simulink model "Hospital"  (R2022b)
settings: Solver=VariableStepAuto  StartTime=0.0  StopTime=10.0  RelTol=1e-3
(part 1 of 2)
settings Model: Creator=Stefano  LastModifiedBy=stefanopanzieri
settings SolverCC: AlgebraicLoopSolver=TrustRegion
settings DebuggingCC: UnconnectedInputMsg=warning  UnconnectedOutputMsg=warning  UnconnectedLineMsg=warning  SFMachineParentedDataDiag=warning
settings ModelReferenceCC: EnableRefExpFcnMdlSchedulingChecks=on
settings SFSimCC: CustomCodeUndefinedFunction=UseInterfaceOnly
settings RTWCC: DLArmComputeVersion=19.05

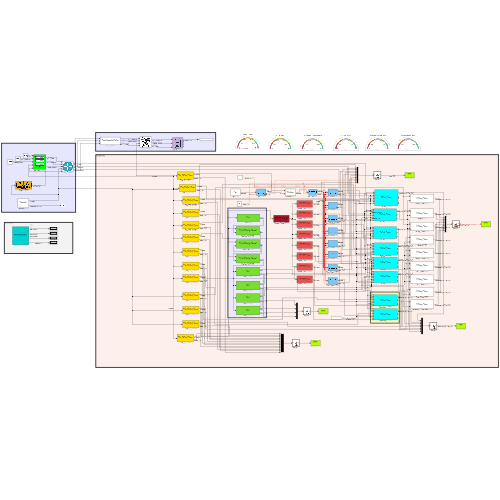
[thumbnail: Simulink's stored preview of the top-level diagram]
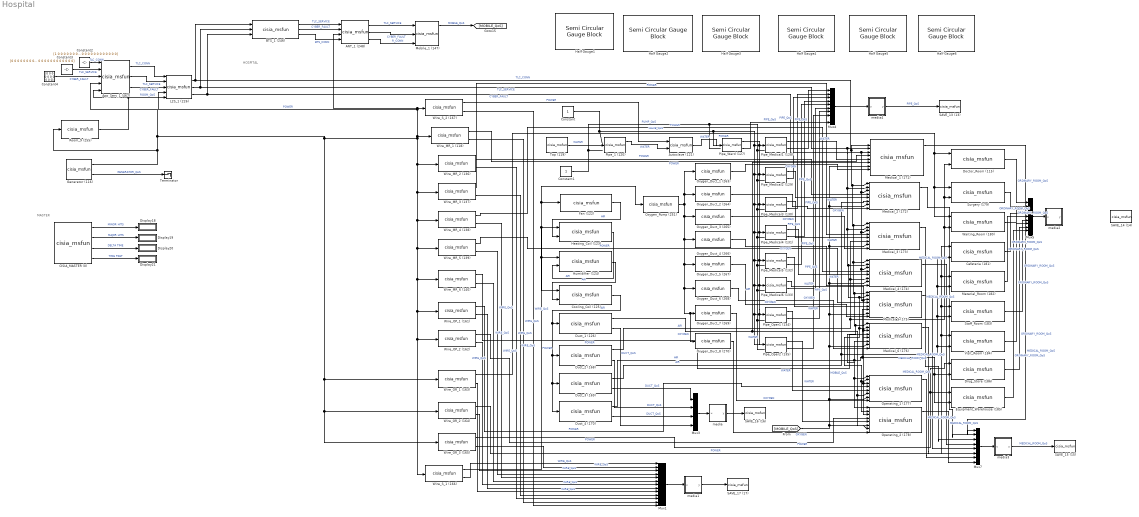
== system Hospital ==
  note: HOSPITAL
  note: MASTER
  ANT_1 (248) : M-S-Function  FunctionName=cisia_msfun  Parameters=Parameter1, Parameter2, Parameter3, resources, Parameter10, codeupdate, step_received, step_computed, dynamic_computed, step_sended, id_entity, id_project, id_type, name_type, color  mask(S-function:msfcn_unit_delay){Parameter1='ANT_1', Parameter2=1, Parameter3='ORO', resources=, Parameter10=off, codeupdate=off, step_received=|, step_computed=, dynamic_computed=, step_sended=|, id_entity=427, id_project=6, id_type=55, name_type=BTS_ANTENNA, color=#FFFFFF}
      mask step_received=|
      | Connection=max(Connection_init,BTS_CONN);
      | TLC_services=max(TLC_services_init,TLC_SERVICE);
      | TLC_services=mod(TLC_services,10);
      | TLC_revoke=floor(TLC_SERVICE/10);
      |
      | Cyber_Fault=max(CYBER_FAULT, transpose([Dos_attack   MITM_attack Virus_Attack Port_Scan_Attack  BGP_hijacking BotNet_Attack Data_Corruption SW_Change Config_Change Port_Saturation]));
      |
      | Conn_Fault=max([Dos_attack  Mechanical_Fault  1-POWER] );
      |
      | Service_Fault=max(abs(Consumed_Services.*TLC_services-Consumed_Services));
      | Redundancy_Fault=max(abs(Consumed_Services.*BTS_CONN-Consumed_Services));
      |
      | Operative_Level=(1-Conn_Fault)*(1-0.5*max(Cyber_Fault))*(1-Service_Fault);
      |
      | %Operative_Level=(1-Conn_Fault)*((2*(1-Service_Fault)+(1-Redundancy_Fault))/3);
      | %Operative_Level=(1-Conn_Fault)*max(max(BTS_CONN),0.5)*((2*(1-Service_Fault)+(1-Redundancy_Fault))/3);
      |
      | % Il servizio utilizzato
      | %My_Service=max([(1-Service_Fault) (1-Redundancy_Fault)/2]);
      mask step_sended=|
      | R_CONN=Connection*(1-Conn_Fault);
      | TLC_SERVICE=TLC_services*(1-Conn_Fault)*(1-Service_Fault)+10*TLC_revoke;
      | CYBER_FAULT=Cyber_Fault*(1-Conn_Fault);
      mask prompts: Parameter1 "entity name"; Parameter2 "sampling time"; Parameter3 "project"; resources "input resources and state variables"; Parameter10 "Bring state variables to output"; codeupdate "update code from mask"
      mask help: This is a level-2 MATLAB file S-function which demonstrates CISIA entity
      mask DialogControl Container1 Prompt: All parameters
      mask Display: image('Icons/BTS_ANTENNA.png')
  App_Serv_1 (467) : M-S-Function  FunctionName=cisia_msfun  Parameters=Parameter1, Parameter2, Parameter3, resources, Parameter10, codeupdate, step_received, step_computed, dynamic_computed, step_sended, id_entity, id_project, id_type, name_type, color  mask(S-function:msfcn_unit_delay){Parameter1='App_Serv_1', Parameter2=1, Parameter3='ORO', resources=, Parameter10=off, codeupdate=off, step_received=|, step_computed=, dynamic_computed=, step_sended=|, id_entity=467, id_project=6, id_type=40, name_type=App_Server, color=#00AAFF}
      mask step_received=|
      | Connection=max(Connection_init,TLC_CONN);
      | TLC_services=max(TLC_services_init,TLC_SERVICE);
      | TLC_services=mod(TLC_services,10);
      | TLC_revoke=floor(TLC_SERVICE/10);
      |
      | Mechanical_Fault=max([Mechanical_Fault Mechanical_Fault_init]);
      |
      | %if strcmp(name_entity,"BlockChainServer") && (cisia.major_time>=2)
      |  % Dos_attack=1;
      |  %TLC_revoke(9)=1;
      |  %TLC_services(9)=0;
      | %end
      |
      |
      | Cyber_Fault=max(CYBER_FAULT, transpose([Dos_attack   MITM_attack Virus_Attack Port_Scan_Attack  BGP_hijacking BotNet_Attack Data_Corruption SW_Change Config_Change Port_Saturation]));
      |
      | Service_Fault=max(abs(Consumed_Services.*TLC_services-Consumed_Services));
      | Redundancy_Fault=max(abs(Consumed_Services.*TLC_CONN-Consumed_Services));
      |
      | Conn_Fault=max([Dos_attack  Mechanical_Fault  1-POWER 1-ROOM_QoS] );
      |
      |
      | Operative_Level=(1-Conn_Fault)*(1-0.5*max(Cyber_Fault))*(1-Service_Fault)*max(max(TLC_CONN),0.5);
      mask step_sended=|
      | TLC_CONN=Connection*(1-Conn_Fault);
      | TLC_SERVICE=TLC_services*(1-Conn_Fault)*(1-Service_Fault)*(1-syslog_adm_login)+10*TLC_revoke;
      | CYBER_FAULT=Cyber_Fault*(1-Conn_Fault);
      mask prompts: Parameter1 "entity name"; Parameter2 "sampling time"; Parameter3 "project"; resources "input resources and state variables"; Parameter10 "Bring state variables to output"; codeupdate "update code from mask"
      mask help: This is a level-2 MATLAB file S-function which demonstrates CISIA entity
      mask DialogControl Container1 Prompt: All parameters
      mask Display: image('Icons/App_Server.png')
  Autoclave (121) : M-S-Function  FunctionName=cisia_msfun  Parameters=Parameter1, Parameter2, Parameter3, resources, Parameter10, codeupdate, step_received, step_computed, dynamic_computed, step_sended, id_entity, id_project, id_type, name_type, color  mask(S-function:msfcn_unit_delay){Parameter1='Autoclave', Parameter2=1, Parameter3='ORO', resources=, Parameter10=off, codeupdate=off, step_received=|, step_computed=, dynamic_computed=, step_sended=WATER=Operative_Level;, id_entity=425, id_project=6, id_type=33, name_type=Autoclave, color=#FFFFFF}
      mask step_received=|
      | Water_Fault=1-WATER;
      | Power_Fault=1-POWER;
      |
      | Operative_Level=min([ 1-Mechanical_Fault 1-Power_Fault 1-Water_Fault]);
      mask prompts: Parameter1 "entity name"; Parameter2 "sampling time"; Parameter3 "project"; resources "input resources and state variables"; Parameter10 "Bring state variables to output"; codeupdate "update code from mask"
      mask help: This is a level-2 MATLAB file S-function which demonstrates CISIA entity
      mask DialogControl Container1 Prompt: All parameters
      mask Display: disp('Autoclave')
  BTS_1 (246) : M-S-Function  FunctionName=cisia_msfun  Parameters=Parameter1, Parameter2, Parameter3, resources, Parameter10, codeupdate, step_received, step_computed, dynamic_computed, step_sended, id_entity, id_project, id_type, name_type, color  mask(S-function:msfcn_unit_delay){Parameter1='BTS_1', Parameter2=1, Parameter3='ORO', resources=, Parameter10=off, codeupdate=off, step_received=|, step_computed=, dynamic_computed=, step_sended=|, id_entity=428, id_project=6, id_type=54, name_type=BaseTransceiverStation, color=#FFFFFF}
      mask step_received=|
      | Connection=max(Connection_init,TLC_CONN);
      | TLC_services=max(TLC_services_init,TLC_SERVICE);
      | TLC_services=mod(TLC_services,10);
      | TLC_revoke=floor(TLC_SERVICE/10);
      |
      | Cyber_Fault=max(CYBER_FAULT, transpose([Dos_attack   MITM_attack Virus_Attack Port_Scan_Attack  BGP_hijacking BotNet_Attack Data_Corruption SW_Change Config_Change Port_Saturation]));
      |
      | Conn_Fault=max([Dos_attack  Mechanical_Fault ] );
      |
      | Operative_Level=(1-Conn_Fault)*max(max(TLC_services),0.5)*(1-0.5*max(Cyber_Fault));
      mask step_sended=|
      | BTS_CONN=Connection*(1-Conn_Fault);
      | TLC_SERVICE=TLC_services*(1-Conn_Fault)+10*TLC_revoke;
      | CYBER_FAULT=Cyber_Fault*(1-Conn_Fault);
      mask prompts: Parameter1 "entity name"; Parameter2 "sampling time"; Parameter3 "project"; resources "input resources and state variables"; Parameter10 "Bring state variables to output"; codeupdate "update code from mask"
      mask help: This is a level-2 MATLAB file S-function which demonstrates CISIA entity
      mask DialogControl Container1 Prompt: All parameters
      mask Display: disp('BaseTransceiverStation')
  CISIA_MASTER (0) : M-S-Function  FunctionName=cisia_msfun  Parameters=Parameter1, Parameter2, Parameter3, resources, Parameter4, Parameter5, Parameter6, Parameter7, Parameter8, Parameter9,Parameter11  mask(S-function:msfcn_unit_delay){Parameter1='CISIA_MASTER', Parameter2=1, Parameter3='SistemiIoT', resources=off, Parameter4=on, Parameter5=off, Parameter6=off, Parameter7=off, Parameter8=0.001, Parameter9=off, Parameter11=on}
      mask prompts: Parameter1 "entity name"; Parameter2 "sampling time"; Parameter3 "project"; resources "Save status at each major hit"; Parameter4 "Show Operative Levels with colors"; Parameter5 "Load Entities from file"; Parameter6 "Load Start from Mask"; Parameter7 "Real Time"; Parameter8 "Real Time Hit (sec)"; Parameter9 "Skip saving"; Parameter11 "Show unconnected"
      mask help: This is a level-2 MATLAB file S-function which demonstrates CISIA entity
      mask Display: disp('MASTER BLOCK')
  Cafeteria (181) : M-S-Function  FunctionName=cisia_msfun  Parameters=Parameter1, Parameter2, Parameter3, resources, Parameter10, codeupdate, step_received, step_computed, dynamic_computed, step_sended, id_entity, id_project, id_type, name_type, color  mask(S-function:msfcn_unit_delay){Parameter1='Cafeteria', Parameter2=1, Parameter3='ORO', resources=, Parameter10=off, codeupdate=off, step_received=|, step_computed=, dynamic_computed=, step_sended=ORDINARY_ROOM_QoS= Operative_Level;, id_entity=385, id_project=6, id_type=26, name_type=Ordinary_Room, color=#FFFFFF}
      mask step_received=|
      | Power_Fault=1-POWER;
      | Air_Fault=1-AIR;
      |
      |
      | Operative_Level=(1-Fire_Fault)*(1-0.5*Power_Fault)*(1-0-5*Air_Fault);
      mask prompts: Parameter1 "entity name"; Parameter2 "sampling time"; Parameter3 "project"; resources "input resources and state variables"; Parameter10 "Bring state variables to output"; codeupdate "update code from mask"
      mask help: This is a level-2 MATLAB file S-function which demonstrates CISIA entity
      mask DialogControl Container1 Prompt: All parameters
      mask Display: disp('Ordinary_Room')
  Constant : Constant
  Constant1 : Constant
  Constant2 : Constant  Value=[1 0 0 0 0 0 0 0 0 0 0 0 0 0 0 0 0 0 0 0]
  Constant3 : Constant  Value=[0 0 0 0 0 0 0 0 0 0 0 0 0 0 0 0 0 0 0 0]
  Constant4 : Constant  Value=[0 0 0 0 0 0 0 0 0 0]
  Cooling_Coil (125) : M-S-Function  FunctionName=cisia_msfun  Parameters=Parameter1, Parameter2, Parameter3, resources, Parameter10, codeupdate, step_received, step_computed, dynamic_computed, step_sended, id_entity, id_project, id_type, name_type, color  mask(S-function:msfcn_unit_delay){Parameter1='Cooling_Coil', Parameter2=1, Parameter3='ORO', resources=, Parameter10=off, codeupdate=off, step_received=|, step_computed=, dynamic_computed=, step_sended=AIR=Operative_Level;, id_entity=395, id_project=6, id_type=35, name_type=Air_Conditioning_Element, color=#79DE31}
      mask step_received=|
      | Power_Fault=1-POWER;
      | Air_Fault=1-AIR;
      |
      | Operative_Level=min([1-Mechanical_Fault 1-Power_Fault 1-Air_Fault]);
      mask prompts: Parameter1 "entity name"; Parameter2 "sampling time"; Parameter3 "project"; resources "input resources and state variables"; Parameter10 "Bring state variables to output"; codeupdate "update code from mask"
      mask help: This is a level-2 MATLAB file S-function which demonstrates CISIA entity
      mask DialogControl Container1 Prompt: All parameters
      mask Display: disp('Air_Conditioning_Element')
  Display{18..21} (4 alike) : Display
  Doctor_Room (115) : M-S-Function  FunctionName=cisia_msfun  Parameters=Parameter1, Parameter2, Parameter3, resources, Parameter10, codeupdate, step_received, step_computed, dynamic_computed, step_sended, id_entity, id_project, id_type, name_type, color  mask(S-function:msfcn_unit_delay){Parameter1='Doctor_Room', Parameter2=1, Parameter3='ORO', resources=, Parameter10=off, codeupdate=off, step_received=|, step_computed=, dynamic_computed=, step_sended=ORDINARY_ROOM_QoS= Operative_Level;, id_entity=414, id_project=6, id_type=26, name_type=Ordinary_Room, color=#FFFFFF}
      mask step_received=|
      | Power_Fault=1-POWER;
      | Air_Fault=1-AIR;
      |
      |
      | Operative_Level=(1-Fire_Fault)*(1-0.5*Power_Fault)*(1-0-5*Air_Fault);
      mask prompts: Parameter1 "entity name"; Parameter2 "sampling time"; Parameter3 "project"; resources "input resources and state variables"; Parameter10 "Bring state variables to output"; codeupdate "update code from mask"
      mask help: This is a level-2 MATLAB file S-function which demonstrates CISIA entity
      mask DialogControl Container1 Prompt: All parameters
      mask Display: disp('Ordinary_Room')
  Drug_Store (186) : M-S-Function  FunctionName=cisia_msfun  Parameters=Parameter1, Parameter2, Parameter3, resources, Parameter10, codeupdate, step_received, step_computed, dynamic_computed, step_sended, id_entity, id_project, id_type, name_type, color  mask(S-function:msfcn_unit_delay){Parameter1='Drug_Store', Parameter2=1, Parameter3='ORO', resources=, Parameter10=off, codeupdate=off, step_received=|, step_computed=, dynamic_computed=, step_sended=ORDINARY_ROOM_QoS= Operative_Level;, id_entity=389, id_project=6, id_type=26, name_type=Ordinary_Room, color=#FFFFFF}
      mask step_received=|
      | Power_Fault=1-POWER;
      | Air_Fault=1-AIR;
      |
      |
      | Operative_Level=(1-Fire_Fault)*(1-0.5*Power_Fault)*(1-0-5*Air_Fault);
      mask prompts: Parameter1 "entity name"; Parameter2 "sampling time"; Parameter3 "project"; resources "input resources and state variables"; Parameter10 "Bring state variables to output"; codeupdate "update code from mask"
      mask help: This is a level-2 MATLAB file S-function which demonstrates CISIA entity
      mask DialogControl Container1 Prompt: All parameters
      mask Display: disp('Ordinary_Room')
  Duct_1 (126) : M-S-Function  FunctionName=cisia_msfun  Parameters=Parameter1, Parameter2, Parameter3, resources, Parameter10, codeupdate, step_received, step_computed, dynamic_computed, step_sended, id_entity, id_project, id_type, name_type, color  mask(S-function:msfcn_unit_delay){Parameter1='Duct_1', Parameter2=1, Parameter3='ORO', resources=, Parameter10=off, codeupdate=off, step_received=|, step_computed=, dynamic_computed=, step_sended=|, id_entity=366, id_project=6, id_type=36, name_type=Duct, color=#79DE31}
      mask step_received=|
      | Air_Fault=1-AIR;
      |
      | Operative_Level=(1-Mechanical_Fault)*(1-0.5*Air_Fault);
      mask step_sended=|
      | AIR=Operative_Level;
      | DUCT_QoS=Operative_Level;
      mask prompts: Parameter1 "entity name"; Parameter2 "sampling time"; Parameter3 "project"; resources "input resources and state variables"; Parameter10 "Bring state variables to output"; codeupdate "update code from mask"
      mask help: This is a level-2 MATLAB file S-function which demonstrates CISIA entity
      mask DialogControl Container1 Prompt: All parameters
      mask Display: disp('Duct')
  Duct_2 (168) : M-S-Function  FunctionName=cisia_msfun  Parameters=Parameter1, Parameter2, Parameter3, resources, Parameter10, codeupdate, step_received, step_computed, dynamic_computed, step_sended, id_entity, id_project, id_type, name_type, color  mask(S-function:msfcn_unit_delay){Parameter1='Duct_2', Parameter2=1, Parameter3='ORO', resources=, Parameter10=off, codeupdate=off, step_received=|, step_computed=, dynamic_computed=, step_sended=|, id_entity=367, id_project=6, id_type=36, name_type=Duct, color=#79DE31}
      mask step_received=|
      | Air_Fault=1-AIR;
      |
      | Operative_Level=(1-Mechanical_Fault)*(1-0.5*Air_Fault);
      mask step_sended=|
      | AIR=Operative_Level;
      | DUCT_QoS=Operative_Level;
      mask prompts: Parameter1 "entity name"; Parameter2 "sampling time"; Parameter3 "project"; resources "input resources and state variables"; Parameter10 "Bring state variables to output"; codeupdate "update code from mask"
      mask help: This is a level-2 MATLAB file S-function which demonstrates CISIA entity
      mask DialogControl Container1 Prompt: All parameters
      mask Display: disp('Duct')
  Duct_3 (169) : M-S-Function  FunctionName=cisia_msfun  Parameters=Parameter1, Parameter2, Parameter3, resources, Parameter10, codeupdate, step_received, step_computed, dynamic_computed, step_sended, id_entity, id_project, id_type, name_type, color  mask(S-function:msfcn_unit_delay){Parameter1='Duct_3', Parameter2=1, Parameter3='ORO', resources=, Parameter10=off, codeupdate=off, step_received=|, step_computed=, dynamic_computed=, step_sended=|, id_entity=368, id_project=6, id_type=36, name_type=Duct, color=#79DE31}
      mask step_received=|
      | Air_Fault=1-AIR;
      |
      | Operative_Level=(1-Mechanical_Fault)*(1-0.5*Air_Fault);
      mask step_sended=|
      | AIR=Operative_Level;
      | DUCT_QoS=Operative_Level;
      mask prompts: Parameter1 "entity name"; Parameter2 "sampling time"; Parameter3 "project"; resources "input resources and state variables"; Parameter10 "Bring state variables to output"; codeupdate "update code from mask"
      mask help: This is a level-2 MATLAB file S-function which demonstrates CISIA entity
      mask DialogControl Container1 Prompt: All parameters
      mask Display: disp('Duct')
  Duct_4 (170) : M-S-Function  FunctionName=cisia_msfun  Parameters=Parameter1, Parameter2, Parameter3, resources, Parameter10, codeupdate, step_received, step_computed, dynamic_computed, step_sended, id_entity, id_project, id_type, name_type, color  mask(S-function:msfcn_unit_delay){Parameter1='Duct_4', Parameter2=1, Parameter3='ORO', resources=, Parameter10=off, codeupdate=off, step_received=|, step_computed=, dynamic_computed=, step_sended=|, id_entity=369, id_project=6, id_type=36, name_type=Duct, color=#79DE31}
      mask step_received=|
      | Air_Fault=1-AIR;
      |
      | Operative_Level=(1-Mechanical_Fault)*(1-0.5*Air_Fault);
      mask step_sended=|
      | AIR=Operative_Level;
      | DUCT_QoS=Operative_Level;
      mask prompts: Parameter1 "entity name"; Parameter2 "sampling time"; Parameter3 "project"; resources "input resources and state variables"; Parameter10 "Bring state variables to output"; codeupdate "update code from mask"
      mask help: This is a level-2 MATLAB file S-function which demonstrates CISIA entity
      mask DialogControl Container1 Prompt: All parameters
      mask Display: disp('Duct')
  Equipment_Warehouse (185) : M-S-Function  FunctionName=cisia_msfun  Parameters=Parameter1, Parameter2, Parameter3, resources, Parameter10, codeupdate, step_received, step_computed, dynamic_computed, step_sended, id_entity, id_project, id_type, name_type, color  mask(S-function:msfcn_unit_delay){Parameter1='Equipment_Warehouse', Parameter2=1, Parameter3='ORO', resources=, Parameter10=off, codeupdate=off, step_received=|, step_computed=, dynamic_computed=, step_sended=ORDINARY_ROOM_QoS= Operative_Level;, id_entity=390, id_project=6, id_type=26, name_type=Ordinary_Room, color=#FFFFFF}
      mask step_received=|
      | Power_Fault=1-POWER;
      | Air_Fault=1-AIR;
      |
      |
      | Operative_Level=(1-Fire_Fault)*(1-0.5*Power_Fault)*(1-0-5*Air_Fault);
      mask prompts: Parameter1 "entity name"; Parameter2 "sampling time"; Parameter3 "project"; resources "input resources and state variables"; Parameter10 "Bring state variables to output"; codeupdate "update code from mask"
      mask help: This is a level-2 MATLAB file S-function which demonstrates CISIA entity
      mask DialogControl Container1 Prompt: All parameters
      mask Display: disp('Ordinary_Room')
  Fan (122) : M-S-Function  FunctionName=cisia_msfun  Parameters=Parameter1, Parameter2, Parameter3, resources, Parameter10, codeupdate, step_received, step_computed, dynamic_computed, step_sended, id_entity, id_project, id_type, name_type, color  mask(S-function:msfcn_unit_delay){Parameter1='Fan', Parameter2=1, Parameter3='ORO', resources=, Parameter10=off, codeupdate=off, step_received=|, step_computed=, dynamic_computed=, step_sended=AIR=Operative_Level;, id_entity=391, id_project=6, id_type=34, name_type=Fan, color=#79DE31}
      mask step_received=|
      | Power_Fault=1-POWER;
      |
      | Operative_Level=(1-Mechanical_Fault)*(1-0.5*Power_Fault);
      mask prompts: Parameter1 "entity name"; Parameter2 "sampling time"; Parameter3 "project"; resources "input resources and state variables"; Parameter10 "Bring state variables to output"; codeupdate "update code from mask"
      mask help: This is a level-2 MATLAB file S-function which demonstrates CISIA entity
      mask DialogControl Container1 Prompt: All parameters
      mask Display: disp('Fan')
  Generator (116) : M-S-Function  FunctionName=cisia_msfun  Parameters=Parameter1, Parameter2, Parameter3, resources, Parameter10, codeupdate, step_received, step_computed, dynamic_computed, step_sended, id_entity, id_project, id_type, name_type, color  mask(S-function:msfcn_unit_delay){Parameter1='Generator', Parameter2=1, Parameter3='ORO', resources=, Parameter10=off, codeupdate=off, step_received=Operative_Level=1-Mechanical_Fault;, step_computed=, dynamic_computed=, step_sended=|, id_entity=392, id_project=6, id_type=27, name_type=Generator, color=#FFFFFF}
      mask step_sended=|
      | POWER=Operative_Level;
      | GENERATOR_QoS=Operative_Level;
      mask prompts: Parameter1 "entity name"; Parameter2 "sampling time"; Parameter3 "project"; resources "input resources and state variables"; Parameter10 "Bring state variables to output"; codeupdate "update code from mask"
      mask help: This is a level-2 MATLAB file S-function which demonstrates CISIA entity
      mask DialogControl Container1 Prompt: All parameters
      mask Display: disp('Generator')
  Half Gauge{1..6} (6 alike) : SemiCircularGaugeBlock  ScaleMax=1
  Heating_Coil (123) : M-S-Function  FunctionName=cisia_msfun  Parameters=Parameter1, Parameter2, Parameter3, resources, Parameter10, codeupdate, step_received, step_computed, dynamic_computed, step_sended, id_entity, id_project, id_type, name_type, color  mask(S-function:msfcn_unit_delay){Parameter1='Heating_Coil', Parameter2=1, Parameter3='ORO', resources=, Parameter10=off, codeupdate=off, step_received=|, step_computed=, dynamic_computed=, step_sended=AIR=Operative_Level;, id_entity=393, id_project=6, id_type=35, name_type=Air_Conditioning_Element, color=#79DE31}
      mask step_received=|
      | Power_Fault=1-POWER;
      | Air_Fault=1-AIR;
      |
      | Operative_Level=min([1-Mechanical_Fault 1-Power_Fault 1-Air_Fault]);
      mask prompts: Parameter1 "entity name"; Parameter2 "sampling time"; Parameter3 "project"; resources "input resources and state variables"; Parameter10 "Bring state variables to output"; codeupdate "update code from mask"
      mask help: This is a level-2 MATLAB file S-function which demonstrates CISIA entity
      mask DialogControl Container1 Prompt: All parameters
      mask Display: disp('Air_Conditioning_Element')
  Humidifier (124) : M-S-Function  FunctionName=cisia_msfun  Parameters=Parameter1, Parameter2, Parameter3, resources, Parameter10, codeupdate, step_received, step_computed, dynamic_computed, step_sended, id_entity, id_project, id_type, name_type, color  mask(S-function:msfcn_unit_delay){Parameter1='Humidifier', Parameter2=1, Parameter3='ORO', resources=, Parameter10=off, codeupdate=off, step_received=|, step_computed=, dynamic_computed=, step_sended=AIR=Operative_Level;, id_entity=394, id_project=6, id_type=35, name_type=Air_Conditioning_Element, color=#79DE31}
      mask step_received=|
      | Power_Fault=1-POWER;
      | Air_Fault=1-AIR;
      |
      | Operative_Level=min([1-Mechanical_Fault 1-Power_Fault 1-Air_Fault]);
      mask prompts: Parameter1 "entity name"; Parameter2 "sampling time"; Parameter3 "project"; resources "input resources and state variables"; Parameter10 "Bring state variables to output"; codeupdate "update code from mask"
      mask help: This is a level-2 MATLAB file S-function which demonstrates CISIA entity
      mask DialogControl Container1 Prompt: All parameters
      mask Display: disp('Air_Conditioning_Element')
  L2S_1 (226) : M-S-Function  FunctionName=cisia_msfun  Parameters=Parameter1, Parameter2, Parameter3, resources, Parameter10, codeupdate, step_received, step_computed, dynamic_computed, step_sended, id_entity, id_project, id_type, name_type, color  mask(S-function:msfcn_unit_delay){Parameter1='L2S_1', Parameter2=1, Parameter3='ORO', resources=, Parameter10=off, codeupdate=off, step_received=|, step_computed=, dynamic_computed=, step_sended=|, id_entity=396, id_project=6, id_type=24, name_type=Layer2Switch, color=#FFFFFF}
      mask step_received=|
      | Connection=max(Connection_init,TLC_CONN);
      | TLC_services=max(TLC_services_init,TLC_SERVICE);
      | TLC_services=mod(TLC_services,10);
      | TLC_revoke=floor(TLC_SERVICE/10);
      |
      | Cyber_Fault=max(CYBER_FAULT, transpose([Dos_attack   MITM_attack Virus_Attack Port_Scan_Attack  BGP_hijacking BotNet_Attack Data_Corruption SW_Change Config_Change Port_Saturation]));
      |
      | Conn_Fault=max([Dos_attack  Mechanical_Fault  1-POWER 1-ROOM_QoS] );
      |
      | Service_Fault=max(abs(Consumed_Services.*TLC_services-Consumed_Services));
      | Redundancy_Fault=max(abs(Consumed_Services.*TLC_CONN-Consumed_Services));
      |
      | Operative_Level=(1-Conn_Fault)*(1-0.5*max(Cyber_Fault))*(1-Service_Fault)*max(max(TLC_CONN),0.5);
      mask step_sended=|
      | TLC_CONN=Connection*(1-Conn_Fault);
      | TLC_SERVICE=TLC_services*(1-Conn_Fault)*(1-Service_Fault)+10*TLC_revoke;
      |
      | Cyber_Transmitted=min(Cyber_Fault, transpose([0 0 1 0 1 1 0 0 0 1]));
      | CYBER_FAULT=Cyber_Transmitted*(1-Conn_Fault);
      mask prompts: Parameter1 "entity name"; Parameter2 "sampling time"; Parameter3 "project"; resources "input resources and state variables"; Parameter10 "Bring state variables to output"; codeupdate "update code from mask"
      mask help: This is a level-2 MATLAB file S-function which demonstrates CISIA entity
      mask DialogControl Container1 Prompt: All parameters
      mask Display: image('Icons/Layer2Switch.png')
  Material_Room (182) : M-S-Function  FunctionName=cisia_msfun  Parameters=Parameter1, Parameter2, Parameter3, resources, Parameter10, codeupdate, step_received, step_computed, dynamic_computed, step_sended, id_entity, id_project, id_type, name_type, color  mask(S-function:msfcn_unit_delay){Parameter1='Material_Room', Parameter2=1, Parameter3='ORO', resources=, Parameter10=off, codeupdate=off, step_received=|, step_computed=, dynamic_computed=, step_sended=ORDINARY_ROOM_QoS= Operative_Level;, id_entity=386, id_project=6, id_type=26, name_type=Ordinary_Room, color=#FFFFFF}
      mask step_received=|
      | Power_Fault=1-POWER;
      | Air_Fault=1-AIR;
      |
      |
      | Operative_Level=(1-Fire_Fault)*(1-0.5*Power_Fault)*(1-0-5*Air_Fault);
      mask prompts: Parameter1 "entity name"; Parameter2 "sampling time"; Parameter3 "project"; resources "input resources and state variables"; Parameter10 "Bring state variables to output"; codeupdate "update code from mask"
      mask help: This is a level-2 MATLAB file S-function which demonstrates CISIA entity
      mask DialogControl Container1 Prompt: All parameters
      mask Display: disp('Ordinary_Room')
  Medical_1 (171) : M-S-Function  FunctionName=cisia_msfun  Parameters=Parameter1, Parameter2, Parameter3, resources, Parameter10, codeupdate, step_received, step_computed, dynamic_computed, step_sended, id_entity, id_project, id_type, name_type, color  mask(S-function:msfcn_unit_delay){Parameter1='Medical_1', Parameter2=1, Parameter3='ORO', resources=, Parameter10=off, codeupdate=off, step_received=|, step_computed=, dynamic_computed=, step_sended=MEDICAL_ROOM_QoS=Operative_Level;, id_entity=397, id_project=6, id_type=25, name_type=Medical_Room, color=#00FFFF}
      mask step_received=|
      | Connection=max(Connection_init,TLC_CONN);
      | TLC_services=max(TLC_services_init,TLC_SERVICE);
      | TLC_services=mod(TLC_services,10);
      | TLC_revoke=floor(TLC_SERVICE/10);
      |
      | Conn_Fault=max([Power_Fault 1-POWER 1-MOBILE_QoS]);
      |
      | Water_Fault=1-WATER;
      | Air_Fault=1-AIR;
      | Physical_Fault=max([Water_Fault Air_Fault 1-OXYGEN]);
      |
      | Service_Fault=max(abs(Consumed_Services.*TLC_services-Consumed_Services));
      | Redundancy_Fault=max(abs(Consumed_Services.*TLC_CONN-Consumed_Services));
      |
      | Operative_Level=(1-Conn_Fault)*(1-0.5*Physical_Fault)*(1-0.5*Service_Fault);
      mask prompts: Parameter1 "entity name"; Parameter2 "sampling time"; Parameter3 "project"; resources "input resources and state variables"; Parameter10 "Bring state variables to output"; codeupdate "update code from mask"
      mask help: This is a level-2 MATLAB file S-function which demonstrates CISIA entity
      mask DialogControl Container1 Prompt: All parameters
      mask Display: disp('Medical_Room')
  Medical_2 (172) : M-S-Function  FunctionName=cisia_msfun  Parameters=Parameter1, Parameter2, Parameter3, resources, Parameter10, codeupdate, step_received, step_computed, dynamic_computed, step_sended, id_entity, id_project, id_type, name_type, color  mask(S-function:msfcn_unit_delay){Parameter1='Medical_2', Parameter2=1, Parameter3='ORO', resources=, Parameter10=off, codeupdate=off, step_received=|, step_computed=, dynamic_computed=, step_sended=MEDICAL_ROOM_QoS=Operative_Level;, id_entity=398, id_project=6, id_type=25, name_type=Medical_Room, color=#00FFFF}
      mask step_received=|
      | Connection=max(Connection_init,TLC_CONN);
      | TLC_services=max(TLC_services_init,TLC_SERVICE);
      | TLC_services=mod(TLC_services,10);
      | TLC_revoke=floor(TLC_SERVICE/10);
      |
      | Conn_Fault=max([Power_Fault 1-POWER 1-MOBILE_QoS]);
      |
      | Water_Fault=1-WATER;
      | Air_Fault=1-AIR;
      | Physical_Fault=max([Water_Fault Air_Fault 1-OXYGEN]);
      |
      | Service_Fault=max(abs(Consumed_Services.*TLC_services-Consumed_Services));
      | Redundancy_Fault=max(abs(Consumed_Services.*TLC_CONN-Consumed_Services));
      |
      | Operative_Level=(1-Conn_Fault)*(1-0.5*Physical_Fault)*(1-0.5*Service_Fault);
      mask prompts: Parameter1 "entity name"; Parameter2 "sampling time"; Parameter3 "project"; resources "input resources and state variables"; Parameter10 "Bring state variables to output"; codeupdate "update code from mask"
      mask help: This is a level-2 MATLAB file S-function which demonstrates CISIA entity
      mask DialogControl Container1 Prompt: All parameters
      mask Display: disp('Medical_Room')
  Medical_3 (173) : M-S-Function  FunctionName=cisia_msfun  Parameters=Parameter1, Parameter2, Parameter3, resources, Parameter10, codeupdate, step_received, step_computed, dynamic_computed, step_sended, id_entity, id_project, id_type, name_type, color  mask(S-function:msfcn_unit_delay){Parameter1='Medical_3', Parameter2=1, Parameter3='ORO', resources=, Parameter10=off, codeupdate=off, step_received=|, step_computed=, dynamic_computed=, step_sended=MEDICAL_ROOM_QoS=Operative_Level;, id_entity=399, id_project=6, id_type=25, name_type=Medical_Room, color=#00FFFF}
      mask step_received=|
      | Connection=max(Connection_init,TLC_CONN);
      | TLC_services=max(TLC_services_init,TLC_SERVICE);
      | TLC_services=mod(TLC_services,10);
      | TLC_revoke=floor(TLC_SERVICE/10);
      |
      | Conn_Fault=max([Power_Fault 1-POWER 1-MOBILE_QoS]);
      |
      | Water_Fault=1-WATER;
      | Air_Fault=1-AIR;
      | Physical_Fault=max([Water_Fault Air_Fault 1-OXYGEN]);
      |
      | Service_Fault=max(abs(Consumed_Services.*TLC_services-Consumed_Services));
      | Redundancy_Fault=max(abs(Consumed_Services.*TLC_CONN-Consumed_Services));
      |
      | Operative_Level=(1-Conn_Fault)*(1-0.5*Physical_Fault)*(1-0.5*Service_Fault);
      mask prompts: Parameter1 "entity name"; Parameter2 "sampling time"; Parameter3 "project"; resources "input resources and state variables"; Parameter10 "Bring state variables to output"; codeupdate "update code from mask"
      mask help: This is a level-2 MATLAB file S-function which demonstrates CISIA entity
      mask DialogControl Container1 Prompt: All parameters
      mask Display: disp('Medical_Room')
  Medical_4 (174) : M-S-Function  FunctionName=cisia_msfun  Parameters=Parameter1, Parameter2, Parameter3, resources, Parameter10, codeupdate, step_received, step_computed, dynamic_computed, step_sended, id_entity, id_project, id_type, name_type, color  mask(S-function:msfcn_unit_delay){Parameter1='Medical_4', Parameter2=1, Parameter3='ORO', resources=, Parameter10=off, codeupdate=off, step_received=|, step_computed=, dynamic_computed=, step_sended=MEDICAL_ROOM_QoS=Operative_Level;, id_entity=400, id_project=6, id_type=25, name_type=Medical_Room, color=#00FFFF}
      mask step_received=|
      | Connection=max(Connection_init,TLC_CONN);
      | TLC_services=max(TLC_services_init,TLC_SERVICE);
      | TLC_services=mod(TLC_services,10);
      | TLC_revoke=floor(TLC_SERVICE/10);
      |
      | Conn_Fault=max([Power_Fault 1-POWER 1-MOBILE_QoS]);
      |
      | Water_Fault=1-WATER;
      | Air_Fault=1-AIR;
      | Physical_Fault=max([Water_Fault Air_Fault 1-OXYGEN]);
      |
      | Service_Fault=max(abs(Consumed_Services.*TLC_services-Consumed_Services));
      | Redundancy_Fault=max(abs(Consumed_Services.*TLC_CONN-Consumed_Services));
      |
      | Operative_Level=(1-Conn_Fault)*(1-0.5*Physical_Fault)*(1-0.5*Service_Fault);
      mask prompts: Parameter1 "entity name"; Parameter2 "sampling time"; Parameter3 "project"; resources "input resources and state variables"; Parameter10 "Bring state variables to output"; codeupdate "update code from mask"
      mask help: This is a level-2 MATLAB file S-function which demonstrates CISIA entity
      mask DialogControl Container1 Prompt: All parameters
      mask Display: disp('Medical_Room')
  Medical_5 (175) : M-S-Function  FunctionName=cisia_msfun  Parameters=Parameter1, Parameter2, Parameter3, resources, Parameter10, codeupdate, step_received, step_computed, dynamic_computed, step_sended, id_entity, id_project, id_type, name_type, color  mask(S-function:msfcn_unit_delay){Parameter1='Medical_5', Parameter2=1, Parameter3='ORO', resources=, Parameter10=off, codeupdate=off, step_received=|, step_computed=, dynamic_computed=, step_sended=MEDICAL_ROOM_QoS=Operative_Level;, id_entity=401, id_project=6, id_type=25, name_type=Medical_Room, color=#00FFFF}
      mask step_received=|
      | Connection=max(Connection_init,TLC_CONN);
      | TLC_services=max(TLC_services_init,TLC_SERVICE);
      | TLC_services=mod(TLC_services,10);
      | TLC_revoke=floor(TLC_SERVICE/10);
      |
      | Conn_Fault=max([Power_Fault 1-POWER 1-MOBILE_QoS]);
      |
      | Water_Fault=1-WATER;
      | Air_Fault=1-AIR;
      | Physical_Fault=max([Water_Fault Air_Fault 1-OXYGEN]);
      |
      | Service_Fault=max(abs(Consumed_Services.*TLC_services-Consumed_Services));
      | Redundancy_Fault=max(abs(Consumed_Services.*TLC_CONN-Consumed_Services));
      |
      | Operative_Level=(1-Conn_Fault)*(1-0.5*Physical_Fault)*(1-0.5*Service_Fault);
      mask prompts: Parameter1 "entity name"; Parameter2 "sampling time"; Parameter3 "project"; resources "input resources and state variables"; Parameter10 "Bring state variables to output"; codeupdate "update code from mask"
      mask help: This is a level-2 MATLAB file S-function which demonstrates CISIA entity
      mask DialogControl Container1 Prompt: All parameters
      mask Display: disp('Medical_Room')
  Medical_6 (176) : M-S-Function  FunctionName=cisia_msfun  Parameters=Parameter1, Parameter2, Parameter3, resources, Parameter10, codeupdate, step_received, step_computed, dynamic_computed, step_sended, id_entity, id_project, id_type, name_type, color  mask(S-function:msfcn_unit_delay){Parameter1='Medical_6', Parameter2=1, Parameter3='ORO', resources=, Parameter10=off, codeupdate=off, step_received=|, step_computed=, dynamic_computed=, step_sended=MEDICAL_ROOM_QoS=Operative_Level;, id_entity=402, id_project=6, id_type=25, name_type=Medical_Room, color=#00FFFF}
      mask step_received=|
      | Connection=max(Connection_init,TLC_CONN);
      | TLC_services=max(TLC_services_init,TLC_SERVICE);
      | TLC_services=mod(TLC_services,10);
      | TLC_revoke=floor(TLC_SERVICE/10);
      |
      | Conn_Fault=max([Power_Fault 1-POWER 1-MOBILE_QoS]);
      |
      | Water_Fault=1-WATER;
      | Air_Fault=1-AIR;
      | Physical_Fault=max([Water_Fault Air_Fault 1-OXYGEN]);
      |
      | Service_Fault=max(abs(Consumed_Services.*TLC_services-Consumed_Services));
      | Redundancy_Fault=max(abs(Consumed_Services.*TLC_CONN-Consumed_Services));
      |
      | Operative_Level=(1-Conn_Fault)*(1-0.5*Physical_Fault)*(1-0.5*Service_Fault);
      mask prompts: Parameter1 "entity name"; Parameter2 "sampling time"; Parameter3 "project"; resources "input resources and state variables"; Parameter10 "Bring state variables to output"; codeupdate "update code from mask"
      mask help: This is a level-2 MATLAB file S-function which demonstrates CISIA entity
      mask DialogControl Container1 Prompt: All parameters
      mask Display: disp('Medical_Room')
  Mobile_1 (147) : M-S-Function  FunctionName=cisia_msfun  Parameters=Parameter1, Parameter2, Parameter3, resources, Parameter10, codeupdate, step_received, step_computed, dynamic_computed, step_sended, id_entity, id_project, id_type, name_type, color  mask(S-function:msfcn_unit_delay){Parameter1='Mobile_1', Parameter2=1, Parameter3='ORO', resources=, Parameter10=off, codeupdate=off, step_received=|, step_computed=, dynamic_computed=, step_sended=|, id_entity=429, id_project=6, id_type=39, name_type=MobileUnit, color=#C9ABDB}
      mask step_received=|
      | Connection=max(Connection_init,R_CONN);
      | TLC_services=max(TLC_services_init,TLC_SERVICE);
      | TLC_services=mod(TLC_services,10);
      | TLC_revoke=floor(TLC_SERVICE/10);
      |
      | Service_Fault=max(abs(Consumed_Services.*TLC_services-Consumed_Services));
      | Redundancy_Fault=max(abs(Consumed_Services.*R_CONN-Consumed_Services));
      |
      | Alt_Serv_Fault=max(abs(Alternative_Services.*R_CONN-Alternative_Services));
      |
      | Alt_Rout_Fault=max(abs(Consumed_Services.*R_CONN-Consumed_Services));
      |
      | Port_Isolation=min(max(transpose([1 1 1 1 1 1 1 1 1 0]), CYBER_FAULT));
      |
      |
      | Operative_Level=(1-Mechanical_Fault)*max(max(R_CONN), 0.5)*(((1-Service_Fault)+(1-Redundancy_Fault)+(1-Port_Isolation))/3);
      |
      | Alt_Port_Isol=(1-Mechanical_Fault)*max(max(R_CONN), 0.5)*(((1-Service_Fault)+(1-Redundancy_Fault))/2);
      mask step_sended=|
      | MOBILE_QoS=Operative_Level;
      |
      |
      | ALT_SERVICES=1-Alt_Serv_Fault;
      | ALT_ROUTING=1-Alt_Rout_Fault;
      | ALT_PORT_ISOLATION=Alt_Port_Isol;
      mask prompts: Parameter1 "entity name"; Parameter2 "sampling time"; Parameter3 "project"; resources "input resources and state variables"; Parameter10 "Bring state variables to output"; codeupdate "update code from mask"
      mask help: This is a level-2 MATLAB file S-function which demonstrates CISIA entity
      mask DialogControl Container1 Prompt: All parameters
      mask Display: image('Icons/MobileUnit.png')
  Mux1 : Mux  Inputs=13
  Mux3 : Mux
  Mux4 : Mux  Inputs=10
  Mux5 : Mux  Inputs=9
  Mux7 : Mux  Inputs=8
  Operating_1 (177) : M-S-Function  FunctionName=cisia_msfun  Parameters=Parameter1, Parameter2, Parameter3, resources, Parameter10, codeupdate, step_received, step_computed, dynamic_computed, step_sended, id_entity, id_project, id_type, name_type, color  mask(S-function:msfcn_unit_delay){Parameter1='Operating_1', Parameter2=1, Parameter3='ORO', resources=, Parameter10=off, codeupdate=off, step_received=|, step_computed=, dynamic_computed=, step_sended=MEDICAL_ROOM_QoS=Operative_Level;, id_entity=403, id_project=6, id_type=25, name_type=Medical_Room, color=#00FFFF}
      mask step_received=|
      | Connection=max(Connection_init,TLC_CONN);
      | TLC_services=max(TLC_services_init,TLC_SERVICE);
      | TLC_services=mod(TLC_services,10);
      | TLC_revoke=floor(TLC_SERVICE/10);
      |
      | Conn_Fault=max([Power_Fault 1-POWER 1-MOBILE_QoS]);
      |
      | Water_Fault=1-WATER;
      | Air_Fault=1-AIR;
      | Physical_Fault=max([Water_Fault Air_Fault 1-OXYGEN]);
      |
      | Service_Fault=max(abs(Consumed_Services.*TLC_services-Consumed_Services));
      | Redundancy_Fault=max(abs(Consumed_Services.*TLC_CONN-Consumed_Services));
      |
      | Operative_Level=(1-Conn_Fault)*(1-0.5*Physical_Fault)*(1-0.5*Service_Fault);
      mask prompts: Parameter1 "entity name"; Parameter2 "sampling time"; Parameter3 "project"; resources "input resources and state variables"; Parameter10 "Bring state variables to output"; codeupdate "update code from mask"
      mask help: This is a level-2 MATLAB file S-function which demonstrates CISIA entity
      mask DialogControl Container1 Prompt: All parameters
      mask Display: disp('Medical_Room')
  Operating_2 (178) : M-S-Function  FunctionName=cisia_msfun  Parameters=Parameter1, Parameter2, Parameter3, resources, Parameter10, codeupdate, step_received, step_computed, dynamic_computed, step_sended, id_entity, id_project, id_type, name_type, color  mask(S-function:msfcn_unit_delay){Parameter1='Operating_2', Parameter2=1, Parameter3='ORO', resources=, Parameter10=off, codeupdate=off, step_received=|, step_computed=, dynamic_computed=, step_sended=MEDICAL_ROOM_QoS=Operative_Level;, id_entity=404, id_project=6, id_type=25, name_type=Medical_Room, color=#00FFFF}
      mask step_received=|
      | Connection=max(Connection_init,TLC_CONN);
      | TLC_services=max(TLC_services_init,TLC_SERVICE);
      | TLC_services=mod(TLC_services,10);
      | TLC_revoke=floor(TLC_SERVICE/10);
      |
      | Conn_Fault=max([Power_Fault 1-POWER 1-MOBILE_QoS]);
      |
      | Water_Fault=1-WATER;
      | Air_Fault=1-AIR;
      | Physical_Fault=max([Water_Fault Air_Fault 1-OXYGEN]);
      |
      | Service_Fault=max(abs(Consumed_Services.*TLC_services-Consumed_Services));
      | Redundancy_Fault=max(abs(Consumed_Services.*TLC_CONN-Consumed_Services));
      |
      | Operative_Level=(1-Conn_Fault)*(1-0.5*Physical_Fault)*(1-0.5*Service_Fault);
      mask prompts: Parameter1 "entity name"; Parameter2 "sampling time"; Parameter3 "project"; resources "input resources and state variables"; Parameter10 "Bring state variables to output"; codeupdate "update code from mask"
      mask help: This is a level-2 MATLAB file S-function which demonstrates CISIA entity
      mask DialogControl Container1 Prompt: All parameters
      mask Display: disp('Medical_Room')
  Oxygen_Duct_1 (263) : M-S-Function  FunctionName=cisia_msfun  Parameters=Parameter1, Parameter2, Parameter3, resources, Parameter10, codeupdate, step_received, step_computed, dynamic_computed, step_sended, id_entity, id_project, id_type, name_type, color  mask(S-function:msfcn_unit_delay){Parameter1='Oxygen_Duct_1', Parameter2=1, Parameter3='ORO', resources=, Parameter10=off, codeupdate=off, step_received=Operative_Level=(1-Mechanical_Fault)*(1-0.5*(1-OXYGEN));, step_computed=, dynamic_computed=, step_sended=OXYGEN=Operative_Level;, id_entity=415, id_project=6, id_type=57, name_type=OXYGEN_Duct, color=#E85151}
      mask prompts: Parameter1 "entity name"; Parameter2 "sampling time"; Parameter3 "project"; resources "input resources and state variables"; Parameter10 "Bring state variables to output"; codeupdate "update code from mask"
      mask help: This is a level-2 MATLAB file S-function which demonstrates CISIA entity
      mask DialogControl Container1 Prompt: All parameters
      mask Display: disp('OXYGEN_Duct')
  Oxygen_Duct_2 (264) : M-S-Function  FunctionName=cisia_msfun  Parameters=Parameter1, Parameter2, Parameter3, resources, Parameter10, codeupdate, step_received, step_computed, dynamic_computed, step_sended, id_entity, id_project, id_type, name_type, color  mask(S-function:msfcn_unit_delay){Parameter1='Oxygen_Duct_2', Parameter2=1, Parameter3='ORO', resources=, Parameter10=off, codeupdate=off, step_received=Operative_Level=(1-Mechanical_Fault)*(1-0.5*(1-OXYGEN));, step_computed=, dynamic_computed=, step_sended=OXYGEN=Operative_Level;, id_entity=416, id_project=6, id_type=57, name_type=OXYGEN_Duct, color=#E85151}
      mask prompts: Parameter1 "entity name"; Parameter2 "sampling time"; Parameter3 "project"; resources "input resources and state variables"; Parameter10 "Bring state variables to output"; codeupdate "update code from mask"
      mask help: This is a level-2 MATLAB file S-function which demonstrates CISIA entity
      mask DialogControl Container1 Prompt: All parameters
      mask Display: disp('OXYGEN_Duct')
  Oxygen_Duct_3 (265) : M-S-Function  FunctionName=cisia_msfun  Parameters=Parameter1, Parameter2, Parameter3, resources, Parameter10, codeupdate, step_received, step_computed, dynamic_computed, step_sended, id_entity, id_project, id_type, name_type, color  mask(S-function:msfcn_unit_delay){Parameter1='Oxygen_Duct_3', Parameter2=1, Parameter3='ORO', resources=, Parameter10=off, codeupdate=off, step_received=Operative_Level=(1-Mechanical_Fault)*(1-0.5*(1-OXYGEN));, step_computed=, dynamic_computed=, step_sended=OXYGEN=Operative_Level;, id_entity=417, id_project=6, id_type=57, name_type=OXYGEN_Duct, color=#E85151}
      mask prompts: Parameter1 "entity name"; Parameter2 "sampling time"; Parameter3 "project"; resources "input resources and state variables"; Parameter10 "Bring state variables to output"; codeupdate "update code from mask"
      mask help: This is a level-2 MATLAB file S-function which demonstrates CISIA entity
      mask DialogControl Container1 Prompt: All parameters
      mask Display: disp('OXYGEN_Duct')
  Oxygen_Duct_4 (266) : M-S-Function  FunctionName=cisia_msfun  Parameters=Parameter1, Parameter2, Parameter3, resources, Parameter10, codeupdate, step_received, step_computed, dynamic_computed, step_sended, id_entity, id_project, id_type, name_type, color  mask(S-function:msfcn_unit_delay){Parameter1='Oxygen_Duct_4', Parameter2=1, Parameter3='ORO', resources=, Parameter10=off, codeupdate=off, step_received=Operative_Level=(1-Mechanical_Fault)*(1-0.5*(1-OXYGEN));, step_computed=, dynamic_computed=, step_sended=OXYGEN=Operative_Level;, id_entity=418, id_project=6, id_type=57, name_type=OXYGEN_Duct, color=#E85151}
      mask prompts: Parameter1 "entity name"; Parameter2 "sampling time"; Parameter3 "project"; resources "input resources and state variables"; Parameter10 "Bring state variables to output"; codeupdate "update code from mask"
      mask help: This is a level-2 MATLAB file S-function which demonstrates CISIA entity
      mask DialogControl Container1 Prompt: All parameters
      mask Display: disp('OXYGEN_Duct')
  Oxygen_Duct_5 (267) : M-S-Function  FunctionName=cisia_msfun  Parameters=Parameter1, Parameter2, Parameter3, resources, Parameter10, codeupdate, step_received, step_computed, dynamic_computed, step_sended, id_entity, id_project, id_type, name_type, color  mask(S-function:msfcn_unit_delay){Parameter1='Oxygen_Duct_5', Parameter2=1, Parameter3='ORO', resources=, Parameter10=off, codeupdate=off, step_received=Operative_Level=(1-Mechanical_Fault)*(1-0.5*(1-OXYGEN));, step_computed=, dynamic_computed=, step_sended=OXYGEN=Operative_Level;, id_entity=419, id_project=6, id_type=57, name_type=OXYGEN_Duct, color=#E85151}
      mask prompts: Parameter1 "entity name"; Parameter2 "sampling time"; Parameter3 "project"; resources "input resources and state variables"; Parameter10 "Bring state variables to output"; codeupdate "update code from mask"
      mask help: This is a level-2 MATLAB file S-function which demonstrates CISIA entity
      mask DialogControl Container1 Prompt: All parameters
      mask Display: disp('OXYGEN_Duct')
  Oxygen_Duct_6 (268) : M-S-Function  FunctionName=cisia_msfun  Parameters=Parameter1, Parameter2, Parameter3, resources, Parameter10, codeupdate, step_received, step_computed, dynamic_computed, step_sended, id_entity, id_project, id_type, name_type, color  mask(S-function:msfcn_unit_delay){Parameter1='Oxygen_Duct_6', Parameter2=1, Parameter3='ORO', resources=, Parameter10=off, codeupdate=off, step_received=Operative_Level=(1-Mechanical_Fault)*(1-0.5*(1-OXYGEN));, step_computed=, dynamic_computed=, step_sended=OXYGEN=Operative_Level;, id_entity=420, id_project=6, id_type=57, name_type=OXYGEN_Duct, color=#E85151}
      mask prompts: Parameter1 "entity name"; Parameter2 "sampling time"; Parameter3 "project"; resources "input resources and state variables"; Parameter10 "Bring state variables to output"; codeupdate "update code from mask"
      mask help: This is a level-2 MATLAB file S-function which demonstrates CISIA entity
      mask DialogControl Container1 Prompt: All parameters
      mask Display: disp('OXYGEN_Duct')
  Oxygen_Duct_7 (269) : M-S-Function  FunctionName=cisia_msfun  Parameters=Parameter1, Parameter2, Parameter3, resources, Parameter10, codeupdate, step_received, step_computed, dynamic_computed, step_sended, id_entity, id_project, id_type, name_type, color  mask(S-function:msfcn_unit_delay){Parameter1='Oxygen_Duct_7', Parameter2=1, Parameter3='ORO', resources=, Parameter10=off, codeupdate=off, step_received=Operative_Level=(1-Mechanical_Fault)*(1-0.5*(1-OXYGEN));, step_computed=, dynamic_computed=, step_sended=OXYGEN=Operative_Level;, id_entity=421, id_project=6, id_type=57, name_type=OXYGEN_Duct, color=#E85151}
      mask prompts: Parameter1 "entity name"; Parameter2 "sampling time"; Parameter3 "project"; resources "input resources and state variables"; Parameter10 "Bring state variables to output"; codeupdate "update code from mask"
      mask help: This is a level-2 MATLAB file S-function which demonstrates CISIA entity
      mask DialogControl Container1 Prompt: All parameters
      mask Display: disp('OXYGEN_Duct')
  Oxygen_Duct_8 (270) : M-S-Function  FunctionName=cisia_msfun  Parameters=Parameter1, Parameter2, Parameter3, resources, Parameter10, codeupdate, step_received, step_computed, dynamic_computed, step_sended, id_entity, id_project, id_type, name_type, color  mask(S-function:msfcn_unit_delay){Parameter1='Oxygen_Duct_8', Parameter2=1, Parameter3='ORO', resources=, Parameter10=off, codeupdate=off, step_received=Operative_Level=(1-Mechanical_Fault)*(1-0.5*(1-OXYGEN));, step_computed=, dynamic_computed=, step_sended=OXYGEN=Operative_Level;, id_entity=422, id_project=6, id_type=57, name_type=OXYGEN_Duct, color=#E85151}
      mask prompts: Parameter1 "entity name"; Parameter2 "sampling time"; Parameter3 "project"; resources "input resources and state variables"; Parameter10 "Bring state variables to output"; codeupdate "update code from mask"
      mask help: This is a level-2 MATLAB file S-function which demonstrates CISIA entity
      mask DialogControl Container1 Prompt: All parameters
      mask Display: disp('OXYGEN_Duct')
  Oxygen_Pump (251) : M-S-Function  FunctionName=cisia_msfun  Parameters=Parameter1, Parameter2, Parameter3, resources, Parameter10, codeupdate, step_received, step_computed, dynamic_computed, step_sended, id_entity, id_project, id_type, name_type, color  mask(S-function:msfcn_unit_delay){Parameter1='Oxygen_Pump', Parameter2=1, Parameter3='ORO', resources=, Parameter10=off, codeupdate=off, step_received=|, step_computed=, dynamic_computed=, step_sended=OXYGEN=Operative_Level;, id_entity=426, id_project=6, id_type=56, name_type=OXYGEN_Element, color=#A11326}
      mask step_received=|
      | Power_Fault=(1-POWER);
      | Operative_Level=(1-Mechanical_Fault)*(1-0.5*Power_Fault);
      mask prompts: Parameter1 "entity name"; Parameter2 "sampling time"; Parameter3 "project"; resources "input resources and state variables"; Parameter10 "Bring state variables to output"; codeupdate "update code from mask"
      mask help: This is a level-2 MATLAB file S-function which demonstrates CISIA entity
      mask DialogControl Container1 Prompt: All parameters
      mask Display: disp('OXYGEN_Element')
  Pipe_1 (120) : M-S-Function  FunctionName=cisia_msfun  Parameters=Parameter1, Parameter2, Parameter3, resources, Parameter10, codeupdate, step_received, step_computed, dynamic_computed, step_sended, id_entity, id_project, id_type, name_type, color  mask(S-function:msfcn_unit_delay){Parameter1='Pipe_1', Parameter2=1, Parameter3='ORO', resources=, Parameter10=off, codeupdate=off, step_received=|, step_computed=, dynamic_computed=, step_sended=|, id_entity=335, id_project=6, id_type=84, name_type=Pipe, color=#00FFFF}
      mask step_received=|
      | Water_Fault=max([1-WATER Mechanical_Fault 1-VALVE_QoS 1-PUMP_QoS]);
      |
      | Operative_Level=1-Mechanical_Fault;
      mask step_sended=|
      | WATER=1-Water_Fault;
      | PIPE_QoS=Operative_Level;
      mask prompts: Parameter1 "entity name"; Parameter2 "sampling time"; Parameter3 "project"; resources "input resources and state variables"; Parameter10 "Bring state variables to output"; codeupdate "update code from mask"
      mask help: This is a level-2 MATLAB file S-function which demonstrates CISIA entity
      mask DialogControl Container1 Prompt: All parameters
      mask Display: image('Icons/Pipe.png')
  Pipe_Medical1 (128) : M-S-Function  FunctionName=cisia_msfun  Parameters=Parameter1, Parameter2, Parameter3, resources, Parameter10, codeupdate, step_received, step_computed, dynamic_computed, step_sended, id_entity, id_project, id_type, name_type, color  mask(S-function:msfcn_unit_delay){Parameter1='Pipe_Medical1', Parameter2=1, Parameter3='ORO', resources=, Parameter10=off, codeupdate=off, step_received=|, step_computed=, dynamic_computed=, step_sended=|, id_entity=406, id_project=6, id_type=84, name_type=Pipe, color=#00FFFF}
      mask step_received=|
      | Water_Fault=max([1-WATER Mechanical_Fault 1-VALVE_QoS 1-PUMP_QoS]);
      |
      | Operative_Level=1-Mechanical_Fault;
      mask step_sended=|
      | WATER=1-Water_Fault;
      | PIPE_QoS=Operative_Level;
      mask prompts: Parameter1 "entity name"; Parameter2 "sampling time"; Parameter3 "project"; resources "input resources and state variables"; Parameter10 "Bring state variables to output"; codeupdate "update code from mask"
      mask help: This is a level-2 MATLAB file S-function which demonstrates CISIA entity
      mask DialogControl Container1 Prompt: All parameters
      mask Display: image('Icons/Pipe.png')
  Pipe_Medical2 (129) : M-S-Function  FunctionName=cisia_msfun  Parameters=Parameter1, Parameter2, Parameter3, resources, Parameter10, codeupdate, step_received, step_computed, dynamic_computed, step_sended, id_entity, id_project, id_type, name_type, color  mask(S-function:msfcn_unit_delay){Parameter1='Pipe_Medical2', Parameter2=1, Parameter3='ORO', resources=, Parameter10=off, codeupdate=off, step_received=|, step_computed=, dynamic_computed=, step_sended=|, id_entity=407, id_project=6, id_type=84, name_type=Pipe, color=#00FFFF}
      mask step_received=|
      | Water_Fault=max([1-WATER Mechanical_Fault 1-VALVE_QoS 1-PUMP_QoS]);
      |
      | Operative_Level=1-Mechanical_Fault;
      mask step_sended=|
      | WATER=1-Water_Fault;
      | PIPE_QoS=Operative_Level;
      mask prompts: Parameter1 "entity name"; Parameter2 "sampling time"; Parameter3 "project"; resources "input resources and state variables"; Parameter10 "Bring state variables to output"; codeupdate "update code from mask"
      mask help: This is a level-2 MATLAB file S-function which demonstrates CISIA entity
      mask DialogControl Container1 Prompt: All parameters
      mask Display: image('Icons/Pipe.png')
  Pipe_Medical3 (130) : M-S-Function  FunctionName=cisia_msfun  Parameters=Parameter1, Parameter2, Parameter3, resources, Parameter10, codeupdate, step_received, step_computed, dynamic_computed, step_sended, id_entity, id_project, id_type, name_type, color  mask(S-function:msfcn_unit_delay){Parameter1='Pipe_Medical3', Parameter2=1, Parameter3='ORO', resources=, Parameter10=off, codeupdate=off, step_received=|, step_computed=, dynamic_computed=, step_sended=|, id_entity=408, id_project=6, id_type=84, name_type=Pipe, color=#00FFFF}
      mask step_received=|
      | Water_Fault=max([1-WATER Mechanical_Fault 1-VALVE_QoS 1-PUMP_QoS]);
      |
      | Operative_Level=1-Mechanical_Fault;
      mask step_sended=|
      | WATER=1-Water_Fault;
      | PIPE_QoS=Operative_Level;
      mask prompts: Parameter1 "entity name"; Parameter2 "sampling time"; Parameter3 "project"; resources "input resources and state variables"; Parameter10 "Bring state variables to output"; codeupdate "update code from mask"
      mask help: This is a level-2 MATLAB file S-function which demonstrates CISIA entity
      mask DialogControl Container1 Prompt: All parameters
      mask Display: image('Icons/Pipe.png')
  Pipe_Medical4 (131) : M-S-Function  FunctionName=cisia_msfun  Parameters=Parameter1, Parameter2, Parameter3, resources, Parameter10, codeupdate, step_received, step_computed, dynamic_computed, step_sended, id_entity, id_project, id_type, name_type, color  mask(S-function:msfcn_unit_delay){Parameter1='Pipe_Medical4', Parameter2=1, Parameter3='ORO', resources=, Parameter10=off, codeupdate=off, step_received=|, step_computed=, dynamic_computed=, step_sended=|, id_entity=409, id_project=6, id_type=84, name_type=Pipe, color=#00FFFF}
      mask step_received=|
      | Water_Fault=max([1-WATER Mechanical_Fault 1-VALVE_QoS 1-PUMP_QoS]);
      |
      | Operative_Level=1-Mechanical_Fault;
      mask step_sended=|
      | WATER=1-Water_Fault;
      | PIPE_QoS=Operative_Level;
      mask prompts: Parameter1 "entity name"; Parameter2 "sampling time"; Parameter3 "project"; resources "input resources and state variables"; Parameter10 "Bring state variables to output"; codeupdate "update code from mask"
      mask help: This is a level-2 MATLAB file S-function which demonstrates CISIA entity
      mask DialogControl Container1 Prompt: All parameters
      mask Display: image('Icons/Pipe.png')
  Pipe_Medical5 (132) : M-S-Function  FunctionName=cisia_msfun  Parameters=Parameter1, Parameter2, Parameter3, resources, Parameter10, codeupdate, step_received, step_computed, dynamic_computed, step_sended, id_entity, id_project, id_type, name_type, color  mask(S-function:msfcn_unit_delay){Parameter1='Pipe_Medical5', Parameter2=1, Parameter3='ORO', resources=, Parameter10=off, codeupdate=off, step_received=|, step_computed=, dynamic_computed=, step_sended=|, id_entity=410, id_project=6, id_type=84, name_type=Pipe, color=#00FFFF}
      mask step_received=|
      | Water_Fault=max([1-WATER Mechanical_Fault 1-VALVE_QoS 1-PUMP_QoS]);
      |
      | Operative_Level=1-Mechanical_Fault;
      mask step_sended=|
      | WATER=1-Water_Fault;
      | PIPE_QoS=Operative_Level;
      mask prompts: Parameter1 "entity name"; Parameter2 "sampling time"; Parameter3 "project"; resources "input resources and state variables"; Parameter10 "Bring state variables to output"; codeupdate "update code from mask"
      mask help: This is a level-2 MATLAB file S-function which demonstrates CISIA entity
      mask DialogControl Container1 Prompt: All parameters
      mask Display: image('Icons/Pipe.png')
  Pipe_Medical6 (133) : M-S-Function  FunctionName=cisia_msfun  Parameters=Parameter1, Parameter2, Parameter3, resources, Parameter10, codeupdate, step_received, step_computed, dynamic_computed, step_sended, id_entity, id_project, id_type, name_type, color  mask(S-function:msfcn_unit_delay){Parameter1='Pipe_Medical6', Parameter2=1, Parameter3='ORO', resources=, Parameter10=off, codeupdate=off, step_received=|, step_computed=, dynamic_computed=, step_sended=|, id_entity=411, id_project=6, id_type=84, name_type=Pipe, color=#00FFFF}
      mask step_received=|
      | Water_Fault=max([1-WATER Mechanical_Fault 1-VALVE_QoS 1-PUMP_QoS]);
      |
      | Operative_Level=1-Mechanical_Fault;
      mask step_sended=|
      | WATER=1-Water_Fault;
      | PIPE_QoS=Operative_Level;
      mask prompts: Parameter1 "entity name"; Parameter2 "sampling time"; Parameter3 "project"; resources "input resources and state variables"; Parameter10 "Bring state variables to output"; codeupdate "update code from mask"
      mask help: This is a level-2 MATLAB file S-function which demonstrates CISIA entity
      mask DialogControl Container1 Prompt: All parameters
      mask Display: image('Icons/Pipe.png')
  Pipe_Oper1 (134) : M-S-Function  FunctionName=cisia_msfun  Parameters=Parameter1, Parameter2, Parameter3, resources, Parameter10, codeupdate, step_received, step_computed, dynamic_computed, step_sended, id_entity, id_project, id_type, name_type, color  mask(S-function:msfcn_unit_delay){Parameter1='Pipe_Oper1', Parameter2=1, Parameter3='ORO', resources=, Parameter10=off, codeupdate=off, step_received=|, step_computed=, dynamic_computed=, step_sended=|, id_entity=412, id_project=6, id_type=84, name_type=Pipe, color=#00FFFF}
      mask step_received=|
      | Water_Fault=max([1-WATER Mechanical_Fault 1-VALVE_QoS 1-PUMP_QoS]);
      |
      | Operative_Level=1-Mechanical_Fault;
      mask step_sended=|
      | WATER=1-Water_Fault;
      | PIPE_QoS=Operative_Level;
      mask prompts: Parameter1 "entity name"; Parameter2 "sampling time"; Parameter3 "project"; resources "input resources and state variables"; Parameter10 "Bring state variables to output"; codeupdate "update code from mask"
      mask help: This is a level-2 MATLAB file S-function which demonstrates CISIA entity
      mask DialogControl Container1 Prompt: All parameters
      mask Display: image('Icons/Pipe.png')
  Pipe_Oper2 (135) : M-S-Function  FunctionName=cisia_msfun  Parameters=Parameter1, Parameter2, Parameter3, resources, Parameter10, codeupdate, step_received, step_computed, dynamic_computed, step_sended, id_entity, id_project, id_type, name_type, color  mask(S-function:msfcn_unit_delay){Parameter1='Pipe_Oper2', Parameter2=1, Parameter3='ORO', resources=, Parameter10=off, codeupdate=off, step_received=|, step_computed=, dynamic_computed=, step_sended=|, id_entity=413, id_project=6, id_type=84, name_type=Pipe, color=#00FFFF}
      mask step_received=|
      | Water_Fault=max([1-WATER Mechanical_Fault 1-VALVE_QoS 1-PUMP_QoS]);
      |
      | Operative_Level=1-Mechanical_Fault;
      mask step_sended=|
      | WATER=1-Water_Fault;
      | PIPE_QoS=Operative_Level;
      mask prompts: Parameter1 "entity name"; Parameter2 "sampling time"; Parameter3 "project"; resources "input resources and state variables"; Parameter10 "Bring state variables to output"; codeupdate "update code from mask"
      mask help: This is a level-2 MATLAB file S-function which demonstrates CISIA entity
      mask DialogControl Container1 Prompt: All parameters
      mask Display: image('Icons/Pipe.png')
  Pipe_Ward (127) : M-S-Function  FunctionName=cisia_msfun  Parameters=Parameter1, Parameter2, Parameter3, resources, Parameter10, codeupdate, step_received, step_computed, dynamic_computed, step_sended, id_entity, id_project, id_type, name_type, color  mask(S-function:msfcn_unit_delay){Parameter1='Pipe_Ward', Parameter2=1, Parameter3='ORO', resources=, Parameter10=off, codeupdate=off, step_received=|, step_computed=, dynamic_computed=, step_sended=|, id_entity=405, id_project=6, id_type=84, name_type=Pipe, color=#00FFFF}
      mask step_received=|
      | Water_Fault=max([1-WATER Mechanical_Fault 1-VALVE_QoS 1-PUMP_QoS]);
      |
      | Operative_Level=1-Mechanical_Fault;
      mask step_sended=|
      | WATER=1-Water_Fault;
      | PIPE_QoS=Operative_Level;
      mask prompts: Parameter1 "entity name"; Parameter2 "sampling time"; Parameter3 "project"; resources "input resources and state variables"; Parameter10 "Bring state variables to output"; codeupdate "update code from mask"
      mask help: This is a level-2 MATLAB file S-function which demonstrates CISIA entity
      mask DialogControl Container1 Prompt: All parameters
      mask Display: image('Icons/Pipe.png')
  Room_9 (255) : M-S-Function  FunctionName=cisia_msfun  Parameters=Parameter1, Parameter2, Parameter3, resources, Parameter10, codeupdate, step_received, step_computed, dynamic_computed, step_sended, id_entity, id_project, id_type, name_type, color  mask(S-function:msfcn_unit_delay){Parameter1='Room_9', Parameter2=1, Parameter3='ORO', resources=, Parameter10=off, codeupdate=off, step_received=|, step_computed=, dynamic_computed=, step_sended=ROOM_QoS=Operative_Level;, id_entity=424, id_project=6, id_type=9, name_type=Room, color=#EDB120}
      mask step_received=|
      | Physical_Fault=max([Power_Fault Flooding_Fault Fire_Fault Cooling_Fault 1-POWER]);
      |
      |
      | %Operative_Level=min([1-Power_Fault 1-Flooding_Fault  1-Fire_Fault  1-Cooling_Fault  POWER]);
      | %Operative_Level=Operative_Level*max((1-Unauthorized_Access),0.5);
      |
      | Operative_Level=(1-Physical_Fault)*(1-0.5*Unauthorized_Access);
      mask prompts: Parameter1 "entity name"; Parameter2 "sampling time"; Parameter3 "project"; resources "input resources and state variables"; Parameter10 "Bring state variables to output"; codeupdate "update code from mask"
      mask help: This is a level-2 MATLAB file S-function which demonstrates CISIA entity
      mask DialogControl Container1 Prompt: All parameters
      mask Display: image('Icons/Room.png')
  SAVE_13 (13) : M-S-Function  FunctionName=cisia_msfun  Parameters=Parameter1, Parameter2, Parameter3  mask(S-function:msfcn_unit_delay){Parameter1='SAVE_13', Parameter2=1, Parameter3='ORO'}
      mask prompts: Parameter1 "entity name"; Parameter2 "sampling time"; Parameter3 "project"
      mask help: This is a level-2 MATLAB file S-function which demonstrates CISIA entity
      mask Display: disp('SAVE')
  SAVE_14 (14) : M-S-Function  FunctionName=cisia_msfun  Parameters=Parameter1, Parameter2, Parameter3  mask(S-function:msfcn_unit_delay){Parameter1='SAVE_14', Parameter2=1, Parameter3='ORO'}
      mask prompts: Parameter1 "entity name"; Parameter2 "sampling time"; Parameter3 "project"
      mask help: This is a level-2 MATLAB file S-function which demonstrates CISIA entity
      mask Display: disp('SAVE')
  SAVE_15 (15) : M-S-Function  FunctionName=cisia_msfun  Parameters=Parameter1, Parameter2, Parameter3  mask(S-function:msfcn_unit_delay){Parameter1='SAVE_15', Parameter2=1, Parameter3='ORO'}
      mask prompts: Parameter1 "entity name"; Parameter2 "sampling time"; Parameter3 "project"
      mask help: This is a level-2 MATLAB file S-function which demonstrates CISIA entity
      mask Display: disp('SAVE')
  SAVE_16 (16) : M-S-Function  FunctionName=cisia_msfun  Parameters=Parameter1, Parameter2, Parameter3  mask(S-function:msfcn_unit_delay){Parameter1='SAVE_16', Parameter2=1, Parameter3='ORO'}
      mask prompts: Parameter1 "entity name"; Parameter2 "sampling time"; Parameter3 "project"
      mask help: This is a level-2 MATLAB file S-function which demonstrates CISIA entity
      mask Display: disp('SAVE')
  SAVE_17 (17) : M-S-Function  FunctionName=cisia_msfun  Parameters=Parameter1, Parameter2, Parameter3  mask(S-function:msfcn_unit_delay){Parameter1='SAVE_17', Parameter2=1, Parameter3='ORO'}
      mask prompts: Parameter1 "entity name"; Parameter2 "sampling time"; Parameter3 "project"
      mask help: This is a level-2 MATLAB file S-function which demonstrates CISIA entity
      mask Display: disp('SAVE')
  Staff_Room (183) : M-S-Function  FunctionName=cisia_msfun  Parameters=Parameter1, Parameter2, Parameter3, resources, Parameter10, codeupdate, step_received, step_computed, dynamic_computed, step_sended, id_entity, id_project, id_type, name_type, color  mask(S-function:msfcn_unit_delay){Parameter1='Staff_Room', Parameter2=1, Parameter3='ORO', resources=, Parameter10=off, codeupdate=off, step_received=|, step_computed=, dynamic_computed=, step_sended=ORDINARY_ROOM_QoS= Operative_Level;, id_entity=387, id_project=6, id_type=26, name_type=Ordinary_Room, color=#FFFFFF}
      mask step_received=|
      | Power_Fault=1-POWER;
      | Air_Fault=1-AIR;
      |
      |
      | Operative_Level=(1-Fire_Fault)*(1-0.5*Power_Fault)*(1-0-5*Air_Fault);
      mask prompts: Parameter1 "entity name"; Parameter2 "sampling time"; Parameter3 "project"; resources "input resources and state variables"; Parameter10 "Bring state variables to output"; codeupdate "update code from mask"
      mask help: This is a level-2 MATLAB file S-function which demonstrates CISIA entity
      mask DialogControl Container1 Prompt: All parameters
      mask Display: disp('Ordinary_Room')
  Surgery (179) : M-S-Function  FunctionName=cisia_msfun  Parameters=Parameter1, Parameter2, Parameter3, resources, Parameter10, codeupdate, step_received, step_computed, dynamic_computed, step_sended, id_entity, id_project, id_type, name_type, color  mask(S-function:msfcn_unit_delay){Parameter1='Surgery', Parameter2=1, Parameter3='ORO', resources=, Parameter10=off, codeupdate=off, step_received=|, step_computed=, dynamic_computed=, step_sended=ORDINARY_ROOM_QoS= Operative_Level;, id_entity=383, id_project=6, id_type=26, name_type=Ordinary_Room, color=#FFFFFF}
      mask step_received=|
      | Power_Fault=1-POWER;
      | Air_Fault=1-AIR;
      |
      |
      | Operative_Level=(1-Fire_Fault)*(1-0.5*Power_Fault)*(1-0-5*Air_Fault);
      mask prompts: Parameter1 "entity name"; Parameter2 "sampling time"; Parameter3 "project"; resources "input resources and state variables"; Parameter10 "Bring state variables to output"; codeupdate "update code from mask"
      mask help: This is a level-2 MATLAB file S-function which demonstrates CISIA entity
      mask DialogControl Container1 Prompt: All parameters
      mask Display: disp('Ordinary_Room')
  Tap (119) : M-S-Function  FunctionName=cisia_msfun  Parameters=Parameter1, Parameter2, Parameter3, resources, Parameter10, codeupdate, step_received, step_computed, dynamic_computed, step_sended, id_entity, id_project, id_type, name_type, color  mask(S-function:msfcn_unit_delay){Parameter1='Tap', Parameter2=1, Parameter3='ORO', resources=, Parameter10=off, codeupdate=off, step_received=Operative_Level=1-Mechanical_Fault;, step_computed=, dynamic_computed=, step_sended=WATER=1-Mechanical_Fault;, id_entity=423, id_project=6, id_type=30, name_type=Tap, color=#FFFFFF}
      mask prompts: Parameter1 "entity name"; Parameter2 "sampling time"; Parameter3 "project"; resources "input resources and state variables"; Parameter10 "Bring state variables to output"; codeupdate "update code from mask"
      mask help: This is a level-2 MATLAB file S-function which demonstrates CISIA entity
      mask DialogControl Container1 Prompt: All parameters
      mask Display: disp('Tap')
  Terminator : Terminator
  Visit_Room (184) : M-S-Function  FunctionName=cisia_msfun  Parameters=Parameter1, Parameter2, Parameter3, resources, Parameter10, codeupdate, step_received, step_computed, dynamic_computed, step_sended, id_entity, id_project, id_type, name_type, color  mask(S-function:msfcn_unit_delay){Parameter1='Visit_Room', Parameter2=1, Parameter3='ORO', resources=, Parameter10=off, codeupdate=off, step_received=|, step_computed=, dynamic_computed=, step_sended=ORDINARY_ROOM_QoS= Operative_Level;, id_entity=388, id_project=6, id_type=26, name_type=Ordinary_Room, color=#FFFFFF}
      mask step_received=|
      | Power_Fault=1-POWER;
      | Air_Fault=1-AIR;
      |
      |
      | Operative_Level=(1-Fire_Fault)*(1-0.5*Power_Fault)*(1-0-5*Air_Fault);
      mask prompts: Parameter1 "entity name"; Parameter2 "sampling time"; Parameter3 "project"; resources "input resources and state variables"; Parameter10 "Bring state variables to output"; codeupdate "update code from mask"
      mask help: This is a level-2 MATLAB file S-function which demonstrates CISIA entity
      mask DialogControl Container1 Prompt: All parameters
      mask Display: disp('Ordinary_Room')
  Waiting_Room (180) : M-S-Function  FunctionName=cisia_msfun  Parameters=Parameter1, Parameter2, Parameter3, resources, Parameter10, codeupdate, step_received, step_computed, dynamic_computed, step_sended, id_entity, id_project, id_type, name_type, color  mask(S-function:msfcn_unit_delay){Parameter1='Waiting_Room', Parameter2=1, Parameter3='ORO', resources=, Parameter10=off, codeupdate=off, step_received=|, step_computed=, dynamic_computed=, step_sended=ORDINARY_ROOM_QoS= Operative_Level;, id_entity=384, id_project=6, id_type=26, name_type=Ordinary_Room, color=#FFFFFF}
      mask step_received=|
      | Power_Fault=1-POWER;
      | Air_Fault=1-AIR;
      |
      |
      | Operative_Level=(1-Fire_Fault)*(1-0.5*Power_Fault)*(1-0-5*Air_Fault);
      mask prompts: Parameter1 "entity name"; Parameter2 "sampling time"; Parameter3 "project"; resources "input resources and state variables"; Parameter10 "Bring state variables to output"; codeupdate "update code from mask"
      mask help: This is a level-2 MATLAB file S-function which demonstrates CISIA entity
      mask DialogControl Container1 Prompt: All parameters
      mask Display: disp('Ordinary_Room')
  Wire_MR_1 (118) : M-S-Function  FunctionName=cisia_msfun  Parameters=Parameter1, Parameter2, Parameter3, resources, Parameter10, codeupdate, step_received, step_computed, dynamic_computed, step_sended, id_entity, id_project, id_type, name_type, color  mask(S-function:msfcn_unit_delay){Parameter1='Wire_MR_1', Parameter2=1, Parameter3='ORO', resources=, Parameter10=off, codeupdate=off, step_received=|, step_computed=, dynamic_computed=, step_sended=|, id_entity=370, id_project=6, id_type=29, name_type=Wire_Medical_Room, color=#FFDD00}
      mask step_received=|
      | Power_Fault=1-POWER;
      |
      | Operative_Level = (1-Mechanical_Fault)*(1-0.5*Power_Fault);
      mask step_sended=|
      | POWER=Operative_Level;
      | WIRE_QoS=Operative_Level;
      mask prompts: Parameter1 "entity name"; Parameter2 "sampling time"; Parameter3 "project"; resources "input resources and state variables"; Parameter10 "Bring state variables to output"; codeupdate "update code from mask"
      mask help: This is a level-2 MATLAB file S-function which demonstrates CISIA entity
      mask DialogControl Container1 Prompt: All parameters
      mask Display: disp('Wire_Medical_Room')
  Wire_MR_2 (136) : M-S-Function  FunctionName=cisia_msfun  Parameters=Parameter1, Parameter2, Parameter3, resources, Parameter10, codeupdate, step_received, step_computed, dynamic_computed, step_sended, id_entity, id_project, id_type, name_type, color  mask(S-function:msfcn_unit_delay){Parameter1='Wire_MR_2', Parameter2=1, Parameter3='ORO', resources=, Parameter10=off, codeupdate=off, step_received=|, step_computed=, dynamic_computed=, step_sended=|, id_entity=371, id_project=6, id_type=29, name_type=Wire_Medical_Room, color=#FFDD00}
      mask step_received=|
      | Power_Fault=1-POWER;
      |
      | Operative_Level = (1-Mechanical_Fault)*(1-0.5*Power_Fault);
      mask step_sended=|
      | POWER=Operative_Level;
      | WIRE_QoS=Operative_Level;
      mask prompts: Parameter1 "entity name"; Parameter2 "sampling time"; Parameter3 "project"; resources "input resources and state variables"; Parameter10 "Bring state variables to output"; codeupdate "update code from mask"
      mask help: This is a level-2 MATLAB file S-function which demonstrates CISIA entity
      mask DialogControl Container1 Prompt: All parameters
      mask Display: disp('Wire_Medical_Room')
  Wire_MR_3 (137) : M-S-Function  FunctionName=cisia_msfun  Parameters=Parameter1, Parameter2, Parameter3, resources, Parameter10, codeupdate, step_received, step_computed, dynamic_computed, step_sended, id_entity, id_project, id_type, name_type, color  mask(S-function:msfcn_unit_delay){Parameter1='Wire_MR_3', Parameter2=1, Parameter3='ORO', resources=, Parameter10=off, codeupdate=off, step_received=|, step_computed=, dynamic_computed=, step_sended=|, id_entity=372, id_project=6, id_type=29, name_type=Wire_Medical_Room, color=#FFDD00}
      mask step_received=|
      | Power_Fault=1-POWER;
      |
      | Operative_Level = (1-Mechanical_Fault)*(1-0.5*Power_Fault);
      mask step_sended=|
      | POWER=Operative_Level;
      | WIRE_QoS=Operative_Level;
      mask prompts: Parameter1 "entity name"; Parameter2 "sampling time"; Parameter3 "project"; resources "input resources and state variables"; Parameter10 "Bring state variables to output"; codeupdate "update code from mask"
      mask help: This is a level-2 MATLAB file S-function which demonstrates CISIA entity
      mask DialogControl Container1 Prompt: All parameters
      mask Display: disp('Wire_Medical_Room')
  Wire_MR_4 (138) : M-S-Function  FunctionName=cisia_msfun  Parameters=Parameter1, Parameter2, Parameter3, resources, Parameter10, codeupdate, step_received, step_computed, dynamic_computed, step_sended, id_entity, id_project, id_type, name_type, color  mask(S-function:msfcn_unit_delay){Parameter1='Wire_MR_4', Parameter2=1, Parameter3='ORO', resources=, Parameter10=off, codeupdate=off, step_received=|, step_computed=, dynamic_computed=, step_sended=|, id_entity=373, id_project=6, id_type=29, name_type=Wire_Medical_Room, color=#FFDD00}
      mask step_received=|
      | Power_Fault=1-POWER;
      |
      | Operative_Level = (1-Mechanical_Fault)*(1-0.5*Power_Fault);
      mask step_sended=|
      | POWER=Operative_Level;
      | WIRE_QoS=Operative_Level;
      mask prompts: Parameter1 "entity name"; Parameter2 "sampling time"; Parameter3 "project"; resources "input resources and state variables"; Parameter10 "Bring state variables to output"; codeupdate "update code from mask"
      mask help: This is a level-2 MATLAB file S-function which demonstrates CISIA entity
      mask DialogControl Container1 Prompt: All parameters
      mask Display: disp('Wire_Medical_Room')
  Wire_MR_5 (139) : M-S-Function  FunctionName=cisia_msfun  Parameters=Parameter1, Parameter2, Parameter3, resources, Parameter10, codeupdate, step_received, step_computed, dynamic_computed, step_sended, id_entity, id_project, id_type, name_type, color  mask(S-function:msfcn_unit_delay){Parameter1='Wire_MR_5', Parameter2=1, Parameter3='ORO', resources=, Parameter10=off, codeupdate=off, step_received=|, step_computed=, dynamic_computed=, step_sended=|, id_entity=374, id_project=6, id_type=29, name_type=Wire_Medical_Room, color=#FFDD00}
      mask step_received=|
      | Power_Fault=1-POWER;
      |
      | Operative_Level = (1-Mechanical_Fault)*(1-0.5*Power_Fault);
      mask step_sended=|
      | POWER=Operative_Level;
      | WIRE_QoS=Operative_Level;
      mask prompts: Parameter1 "entity name"; Parameter2 "sampling time"; Parameter3 "project"; resources "input resources and state variables"; Parameter10 "Bring state variables to output"; codeupdate "update code from mask"
      mask help: This is a level-2 MATLAB file S-function which demonstrates CISIA entity
      mask DialogControl Container1 Prompt: All parameters
      mask Display: disp('Wire_Medical_Room')
  Wire_MR_6 (140) : M-S-Function  FunctionName=cisia_msfun  Parameters=Parameter1, Parameter2, Parameter3, resources, Parameter10, codeupdate, step_received, step_computed, dynamic_computed, step_sended, id_entity, id_project, id_type, name_type, color  mask(S-function:msfcn_unit_delay){Parameter1='Wire_MR_6', Parameter2=1, Parameter3='ORO', resources=, Parameter10=off, codeupdate=off, step_received=|, step_computed=, dynamic_computed=, step_sended=|, id_entity=375, id_project=6, id_type=29, name_type=Wire_Medical_Room, color=#FFDD00}
      mask step_received=|
      | Power_Fault=1-POWER;
      |
      | Operative_Level = (1-Mechanical_Fault)*(1-0.5*Power_Fault);
      mask step_sended=|
      | POWER=Operative_Level;
      | WIRE_QoS=Operative_Level;
      mask prompts: Parameter1 "entity name"; Parameter2 "sampling time"; Parameter3 "project"; resources "input resources and state variables"; Parameter10 "Bring state variables to output"; codeupdate "update code from mask"
      mask help: This is a level-2 MATLAB file S-function which demonstrates CISIA entity
      mask DialogControl Container1 Prompt: All parameters
      mask Display: disp('Wire_Medical_Room')
  Wire_OP_1 (161) : M-S-Function  FunctionName=cisia_msfun  Parameters=Parameter1, Parameter2, Parameter3, resources, Parameter10, codeupdate, step_received, step_computed, dynamic_computed, step_sended, id_entity, id_project, id_type, name_type, color  mask(S-function:msfcn_unit_delay){Parameter1='Wire_OP_1', Parameter2=1, Parameter3='ORO', resources=, Parameter10=off, codeupdate=off, step_received=|, step_computed=, dynamic_computed=, step_sended=|, id_entity=376, id_project=6, id_type=29, name_type=Wire_Medical_Room, color=#FFDD00}
      mask step_received=|
      | Power_Fault=1-POWER;
      |
      | Operative_Level = (1-Mechanical_Fault)*(1-0.5*Power_Fault);
      mask step_sended=|
      | POWER=Operative_Level;
      | WIRE_QoS=Operative_Level;
      mask prompts: Parameter1 "entity name"; Parameter2 "sampling time"; Parameter3 "project"; resources "input resources and state variables"; Parameter10 "Bring state variables to output"; codeupdate "update code from mask"
      mask help: This is a level-2 MATLAB file S-function which demonstrates CISIA entity
      mask DialogControl Container1 Prompt: All parameters
      mask Display: disp('Wire_Medical_Room')
  Wire_OP_2 (162) : M-S-Function  FunctionName=cisia_msfun  Parameters=Parameter1, Parameter2, Parameter3, resources, Parameter10, codeupdate, step_received, step_computed, dynamic_computed, step_sended, id_entity, id_project, id_type, name_type, color  mask(S-function:msfcn_unit_delay){Parameter1='Wire_OP_2', Parameter2=1, Parameter3='ORO', resources=, Parameter10=off, codeupdate=off, step_received=|, step_computed=, dynamic_computed=, step_sended=|, id_entity=377, id_project=6, id_type=29, name_type=Wire_Medical_Room, color=#FFDD00}
      mask step_received=|
      | Power_Fault=1-POWER;
      |
      | Operative_Level = (1-Mechanical_Fault)*(1-0.5*Power_Fault);
      mask step_sended=|
      | POWER=Operative_Level;
      | WIRE_QoS=Operative_Level;
      mask prompts: Parameter1 "entity name"; Parameter2 "sampling time"; Parameter3 "project"; resources "input resources and state variables"; Parameter10 "Bring state variables to output"; codeupdate "update code from mask"
      mask help: This is a level-2 MATLAB file S-function which demonstrates CISIA entity
      mask DialogControl Container1 Prompt: All parameters
      mask Display: disp('Wire_Medical_Room')
  Wire_OR_1 (163) : M-S-Function  FunctionName=cisia_msfun  Parameters=Parameter1, Parameter2, Parameter3, resources, Parameter10, codeupdate, step_received, step_computed, dynamic_computed, step_sended, id_entity, id_project, id_type, name_type, color  mask(S-function:msfcn_unit_delay){Parameter1='Wire_OR_1', Parameter2=1, Parameter3='ORO', resources=, Parameter10=off, codeupdate=off, step_received=|, step_computed=, dynamic_computed=, step_sended=|, id_entity=378, id_project=6, id_type=29, name_type=Wire_Medical_Room, color=#FFDD00}
      mask step_received=|
      | Power_Fault=1-POWER;
      |
      | Operative_Level = (1-Mechanical_Fault)*(1-0.5*Power_Fault);
      mask step_sended=|
      | POWER=Operative_Level;
      | WIRE_QoS=Operative_Level;
      mask prompts: Parameter1 "entity name"; Parameter2 "sampling time"; Parameter3 "project"; resources "input resources and state variables"; Parameter10 "Bring state variables to output"; codeupdate "update code from mask"
      mask help: This is a level-2 MATLAB file S-function which demonstrates CISIA entity
      mask DialogControl Container1 Prompt: All parameters
      mask Display: disp('Wire_Medical_Room')
  Wire_OR_2 (164) : M-S-Function  FunctionName=cisia_msfun  Parameters=Parameter1, Parameter2, Parameter3, resources, Parameter10, codeupdate, step_received, step_computed, dynamic_computed, step_sended, id_entity, id_project, id_type, name_type, color  mask(S-function:msfcn_unit_delay){Parameter1='Wire_OR_2', Parameter2=1, Parameter3='ORO', resources=, Parameter10=off, codeupdate=off, step_received=|, step_computed=, dynamic_computed=, step_sended=|, id_entity=379, id_project=6, id_type=29, name_type=Wire_Medical_Room, color=#FFDD00}
      mask step_received=|
      | Power_Fault=1-POWER;
      |
      | Operative_Level = (1-Mechanical_Fault)*(1-0.5*Power_Fault);
      mask step_sended=|
      | POWER=Operative_Level;
      | WIRE_QoS=Operative_Level;
      mask prompts: Parameter1 "entity name"; Parameter2 "sampling time"; Parameter3 "project"; resources "input resources and state variables"; Parameter10 "Bring state variables to output"; codeupdate "update code from mask"
      mask help: This is a level-2 MATLAB file S-function which demonstrates CISIA entity
      mask DialogControl Container1 Prompt: All parameters
      mask Display: disp('Wire_Medical_Room')
  Wire_OR_3 (165) : M-S-Function  FunctionName=cisia_msfun  Parameters=Parameter1, Parameter2, Parameter3, resources, Parameter10, codeupdate, step_received, step_computed, dynamic_computed, step_sended, id_entity, id_project, id_type, name_type, color  mask(S-function:msfcn_unit_delay){Parameter1='Wire_OR_3', Parameter2=1, Parameter3='ORO', resources=, Parameter10=off, codeupdate=off, step_received=|, step_computed=, dynamic_computed=, step_sended=|, id_entity=380, id_project=6, id_type=29, name_type=Wire_Medical_Room, color=#FFDD00}
      mask step_received=|
      | Power_Fault=1-POWER;
      |
      | Operative_Level = (1-Mechanical_Fault)*(1-0.5*Power_Fault);
      mask step_sended=|
      | POWER=Operative_Level;
      | WIRE_QoS=Operative_Level;
      mask prompts: Parameter1 "entity name"; Parameter2 "sampling time"; Parameter3 "project"; resources "input resources and state variables"; Parameter10 "Bring state variables to output"; codeupdate "update code from mask"
      mask help: This is a level-2 MATLAB file S-function which demonstrates CISIA entity
      mask DialogControl Container1 Prompt: All parameters
      mask Display: disp('Wire_Medical_Room')
  Wire_S_1 (166) : M-S-Function  FunctionName=cisia_msfun  Parameters=Parameter1, Parameter2, Parameter3, resources, Parameter10, codeupdate, step_received, step_computed, dynamic_computed, step_sended, id_entity, id_project, id_type, name_type, color  mask(S-function:msfcn_unit_delay){Parameter1='Wire_S_1', Parameter2=1, Parameter3='ORO', resources=, Parameter10=off, codeupdate=off, step_received=|, step_computed=, dynamic_computed=, step_sended=|, id_entity=381, id_project=6, id_type=29, name_type=Wire_Medical_Room, color=#FFDD00}
      mask step_received=|
      | Power_Fault=1-POWER;
      |
      | Operative_Level = (1-Mechanical_Fault)*(1-0.5*Power_Fault);
      mask step_sended=|
      | POWER=Operative_Level;
      | WIRE_QoS=Operative_Level;
      mask prompts: Parameter1 "entity name"; Parameter2 "sampling time"; Parameter3 "project"; resources "input resources and state variables"; Parameter10 "Bring state variables to output"; codeupdate "update code from mask"
      mask help: This is a level-2 MATLAB file S-function which demonstrates CISIA entity
      mask DialogControl Container1 Prompt: All parameters
      mask Display: disp('Wire_Medical_Room')
  Wire_S_2 (167) : M-S-Function  FunctionName=cisia_msfun  Parameters=Parameter1, Parameter2, Parameter3, resources, Parameter10, codeupdate, step_received, step_computed, dynamic_computed, step_sended, id_entity, id_project, id_type, name_type, color  mask(S-function:msfcn_unit_delay){Parameter1='Wire_S_2', Parameter2=1, Parameter3='ORO', resources=, Parameter10=off, codeupdate=off, step_received=|, step_computed=, dynamic_computed=, step_sended=|, id_entity=382, id_project=6, id_type=29, name_type=Wire_Medical_Room, color=#FFDD00}
      mask step_received=|
      | Power_Fault=1-POWER;
      |
      | Operative_Level = (1-Mechanical_Fault)*(1-0.5*Power_Fault);
      mask step_sended=|
      | POWER=Operative_Level;
      | WIRE_QoS=Operative_Level;
      mask prompts: Parameter1 "entity name"; Parameter2 "sampling time"; Parameter3 "project"; resources "input resources and state variables"; Parameter10 "Bring state variables to output"; codeupdate "update code from mask"
      mask help: This is a level-2 MATLAB file S-function which demonstrates CISIA entity
      mask DialogControl Container1 Prompt: All parameters
      mask Display: disp('Wire_Medical_Room')
  media : MATLAB Function  TreatAsAtomicUnit=on
  media1 : MATLAB Function  TreatAsAtomicUnit=on
  media2 : MATLAB Function  TreatAsAtomicUnit=on
  media3 : MATLAB Function  TreatAsAtomicUnit=on
  media4 : MATLAB Function  TreatAsAtomicUnit=on
  wires:
  Wire_OP_1 (161)/1 -> Operating_1 (177)/4  "POWER"
  Humidifier (124)/1 -> Cooling_Coil (125)/2  "AIR"
  Heating_Coil (123)/1 -> Humidifier (124)/2  "AIR"
  Tap (119)/1 -> Pipe_1 (120)/1  "WATER"
  Wire_OR_3 (165)/1 -> Drug_Store (186)/1, Equipment_Warehouse (185)/1  "POWER"
  Wire_MR_4 (138)/1 -> Medical_4 (174)/4  "POWER"
  Duct_2 (168)/1 -> Medical_3 (173)/6, Medical_4 (174)/6, Waiting_Room (180)/2, Surgery (179)/2, Doctor_Room (115)/2  "AIR"
  Pipe_Oper2 (135)/2 -> Mux4/8  "PIPE_QoS"
  Fan (122)/1 -> Heating_Coil (123)/2  "AIR"
  Pipe_Oper1 (134)/1 -> Operating_1 (177)/5  "WATER"
  Pipe_Medical3 (130)/1 -> Medical_3 (173)/5  "WATER"
  Pipe_Oper2 (135)/1 -> Operating_2 (178)/5  "WATER"
  Wire_MR_5 (139)/1 -> Medical_5 (175)/4  "POWER"
  Wire_MR_3 (137)/1 -> Medical_3 (173)/4  "POWER"
  Pipe_Oper1 (134)/2 -> Mux4/7  "PIPE_QoS"
  Wire_MR_3 (137)/2 -> Mux1/10  "WIRE_QoS"
  Pipe_Medical4 (131)/1 -> Medical_4 (174)/5  "WATER"
  Pipe_Medical5 (132)/2 -> Mux4/5  "PIPE_QoS"
  Mux3/1 -> media/1(u)
  Pipe_Medical6 (133)/2 -> Mux4/6  "PIPE_QoS"
  Pipe_Medical2 (129)/2 -> Mux4/3  "PIPE_QoS"
  Pipe_Medical6 (133)/1 -> Medical_6 (176)/5  "WATER"
  Wire_MR_4 (138)/2 -> Mux1/5  "WIRE_QoS"
  Duct_4 (170)/2 -> Mux3/3  "DUCT_QoS"
  ? -> Mux4/9  "PIPE_QoS"
  Pipe_Medical4 (131)/2 -> Mux4/4  "PIPE_QoS"
  Wire_S_1 (166)/2 -> Mux1/1  "WIRE_QoS"
  Wire_S_1 (166)/1 -> Oxygen_Pump (251)/1, Fan (122)/1, Humidifier (124)/1, Cooling_Coil (125)/1, Heating_Coil (123)/1  "POWER"
  Duct_3 (169)/2 -> Mux3/1  "DUCT_QoS"
  Duct_2 (168)/2 -> Mux3/2  "DUCT_QoS"
  Pipe_Medical5 (132)/1 -> Medical_5 (175)/5  "WATER"
  Cooling_Coil (125)/1 -> Duct_4 (170)/1, Duct_3 (169)/1, Duct_2 (168)/1, Duct_1 (126)/1  "AIR"
  Duct_3 (169)/1 -> Medical_2 (172)/6, Visit_Room (184)/2, Staff_Room (183)/2, Material_Room (182)/2, Cafeteria (181)/2  "AIR"
  Pipe_Medical3 (130)/2 -> Mux4/2  "PIPE_QoS"
  Duct_4 (170)/1 -> Medical_6 (176)/6, Medical_5 (175)/6, Equipment_Warehouse (185)/2, Drug_Store (186)/2  "AIR"
  Pipe_Ward (127)/2 -> Mux4/10  "PIPE_QoS"
  Wire_OR_2 (164)/1 -> Visit_Room (184)/1, Staff_Room (183)/1, Material_Room (182)/1, Cafeteria (181)/1  "POWER"
  Wire_MR_6 (140)/1 -> Medical_6 (176)/4  "POWER"
  Wire_MR_5 (139)/2 -> Mux1/4  "WIRE_QoS"
  Autoclave (121)/1 -> Pipe_Ward (127)/1  "WATER"
  Pipe_Medical2 (129)/1 -> Medical_2 (172)/5  "WATER"
  Pipe_Ward (127)/1 -> Pipe_Medical5 (132)/1, Pipe_Oper2 (135)/1, Pipe_Oper1 (134)/1, Pipe_Medical6 (133)/1, Pipe_Medical4 (131)/1, Pipe_Medical3 (130)/1, Pipe_Medical2 (129)/1, Pipe_Medical1 (128)/1  "WATER"
  Wire_MR_6 (140)/2 -> Mux1/6  "WIRE_QoS"
  Wire_MR_2 (136)/1 -> Medical_2 (172)/4  "POWER"
  Pipe_Medical1 (128)/2 -> Mux4/1  "PIPE_QoS"
  Mux4/1 -> media4/1(u)
  Wire_OP_2 (162)/2 -> Mux1/7  "WIRE_QoS"
  Wire_OR_1 (163)/2 -> Mux1/9  "WIRE_QoS"
  Mux1/1 -> media1/1(u)
  Wire_MR_1 (118)/2 -> Mux1/12  "WIRE_QoS"
  Wire_OR_1 (163)/1 -> Waiting_Room (180)/1, Surgery (179)/1, Doctor_Room (115)/1  "POWER"
  Wire_OR_2 (164)/2 -> Mux1/3  "WIRE_QoS"
  Wire_MR_2 (136)/2 -> Mux1/11  "WIRE_QoS"
  Wire_OR_3 (165)/2 -> Mux1/2  "WIRE_QoS"
  Duct_1 (126)/1 -> Operating_2 (178)/6, Operating_1 (177)/6, Medical_1 (171)/6  "AIR"
  Wire_OP_2 (162)/1 -> Operating_2 (178)/4  "POWER"
  Duct_1 (126)/2 -> Mux3/4  "DUCT_QoS"
  L2S_1 (226)/1 -> BTS_1 (246)/1, Medical_1 (171)/1, Operating_2 (178)/1, Operating_1 (177)/1, Medical_6 (176)/1, Medical_5 (175)/1, Medical_4 (174)/1, Medical_3 (173)/1, Medical_2 (172)/1  "TLC_CONN"
  L2S_1 (226)/2 -> BTS_1 (246)/2, Medical_1 (171)/2, Operating_2 (178)/2, Operating_1 (177)/2, Medical_6 (176)/2, Medical_5 (175)/2, Medical_4 (174)/2, Medical_3 (173)/2, Medical_2 (172)/2  "TLC_SERVICE"
  L2S_1 (226)/3 -> BTS_1 (246)/3, Medical_1 (171)/3, Operating_2 (178)/3, Operating_1 (177)/3, Medical_6 (176)/3, Medical_5 (175)/3, Medical_4 (174)/3, Medical_3 (173)/3, Medical_2 (172)/3  "CYBER_FAULT"
  [MOBILE_QoS] -> Medical_1 (171)/7, Medical_2 (172)/7, Medical_3 (173)/7, Medical_4 (174)/7, Medical_5 (175)/7, Medical_6 (176)/7, Operating_1 (177)/7, Operating_2 (178)/7  "MOBILE_QoS"
  media4/1(y) -> SAVE_13 (13)/1  "PIPE_QoS"
  Staff_Room (183)/1 -> Mux5/6  "ORDINARY_ROOM_QoS"
  media/1(y) -> SAVE_16 (16)/1
  media1/1(y) -> SAVE_17 (17)/1
  Room_9 (255)/1 -> App_Serv_1 (467)/5, L2S_1 (226)/5  "ROOM_QoS"
  Doctor_Room (115)/1 -> Mux5/1  "ORDINARY_ROOM_QoS"
  Surgery (179)/1 -> Mux5/2  "ORDINARY_ROOM_QoS"
  Waiting_Room (180)/1 -> Mux5/3  "ORDINARY_ROOM_QoS"
  Cafeteria (181)/1 -> Mux5/4  "ORDINARY_ROOM_QoS"
  Material_Room (182)/1 -> Mux5/5  "ORDINARY_ROOM_QoS"
  Visit_Room (184)/1 -> Mux5/7  "ORDINARY_ROOM_QoS"
  Drug_Store (186)/1 -> Mux5/8  "ORDINARY_ROOM_QoS"
  Equipment_Warehouse (185)/1 -> Mux5/9  "ORDINARY_ROOM_QoS"
  Mux5/1 -> media2/1(u)
  ? -> SAVE_14 (14)/1  "ORDINARY_ROOM_QoS"
  Operating_2 (178)/1 -> Mux7/8  "MEDICAL_ROOM_QoS"
  Operating_1 (177)/1 -> Mux7/7  "MEDICAL_ROOM_QoS"
  Medical_6 (176)/1 -> Mux7/6  "MEDICAL_ROOM_QoS"
  Medical_5 (175)/1 -> Mux7/5  "MEDICAL_ROOM_QoS"
  Medical_4 (174)/1 -> Mux7/4  "MEDICAL_ROOM_QoS"
  Medical_3 (173)/1 -> Mux7/3  "MEDICAL_ROOM_QoS"
  Medical_2 (172)/1 -> Mux7/2  "MEDICAL_ROOM_QoS"
  Medical_1 (171)/1 -> Mux7/1  "MEDICAL_ROOM_QoS"
  Mux7/1 -> media3/1(u)
  media3/1(y) -> SAVE_15 (15)/1  "MEDICAL_ROOM_QoS"
  Oxygen_Pump (251)/1 -> Oxygen_Duct_7 (269)/1, Oxygen_Duct_8 (270)/1, Oxygen_Duct_6 (268)/1, Oxygen_Duct_5 (267)/1, Oxygen_Duct_4 (266)/1, Oxygen_Duct_3 (265)/1, Oxygen_Duct_2 (264)/1, Oxygen_Duct_1 (263)/1  "OXYGEN"
  Oxygen_Duct_2 (264)/1 -> Medical_2 (172)/8  "OXYGEN"
  Oxygen_Duct_3 (265)/1 -> Medical_3 (173)/8  "OXYGEN"
  Oxygen_Duct_4 (266)/1 -> Medical_4 (174)/8  "OXYGEN"
  Oxygen_Duct_5 (267)/1 -> Medical_5 (175)/8  "OXYGEN"
  Oxygen_Duct_6 (268)/1 -> Medical_6 (176)/8  "OXYGEN"
  Oxygen_Duct_7 (269)/1 -> Operating_1 (177)/8  "OXYGEN"
  Oxygen_Duct_8 (270)/1 -> Operating_2 (178)/8  "OXYGEN"
  Wire_OP_1 (161)/2 -> Mux1/8  "WIRE_QoS"
  Pipe_1 (120)/1 -> Autoclave (121)/2  "WATER"
  Wire_S_2 (167)/1 -> Autoclave (121)/1  "POWER"
  Wire_S_2 (167)/2 -> Mux1/13  "WIRE_QoS"
  Wire_MR_1 (118)/1 -> Medical_1 (171)/4  "POWER"
  Pipe_Medical1 (128)/1 -> Medical_1 (171)/5  "WATER"
  Oxygen_Duct_1 (263)/1 -> Medical_1 (171)/8  "OXYGEN"
  ANT_1 (248)/1 -> Mobile_1 (147)/1  "TLC_SERVICE"
  ANT_1 (248)/3 -> Mobile_1 (147)/3  "R_CONN"
  Mobile_1 (147)/1 -> [MOBILE_QoS]  "MOBILE_QoS"
  BTS_1 (246)/2 -> ANT_1 (248)/2  "CYBER_FAULT"
  BTS_1 (246)/1 -> ANT_1 (248)/1  "TLC_SERVICE"
  ANT_1 (248)/2 -> Mobile_1 (147)/2  "CYBER_FAULT"
  Generator (116)/1 -> App_Serv_1 (467)/4, ANT_1 (248)/3, Wire_S_2 (167)/1, L2S_1 (226)/4, Wire_MR_1 (118)/1, Wire_S_1 (166)/1, Wire_OP_2 (162)/1, Wire_OP_1 (161)/1, Wire_MR_6 (140)/1, Wire_MR_5 (139)/1, Wire_MR_4 (138)/1, Wire_MR_3 (137)/1, Wire_MR_2 (136)/1, Wire_OR_3 (165)/1, Wire_OR_2 (164)/1, Wire_OR_1 (163)/1, Room_9 (255)/1  "POWER"
  BTS_1 (246)/3 -> ANT_1 (248)/4  "BTS_CONN"
  Constant/1 -> ?  "VALVE_QoS"
  Constant1/1 -> ?  "PUMP_QoS"
  Generator (116)/2 -> Terminator/1  "GENERATOR_QoS"
  Constant2/1 -> App_Serv_1 (467)/1  "TLC_CONN"
  Constant3/1 -> App_Serv_1 (467)/2  "TLC_SERVICE"
  Constant4/1 -> App_Serv_1 (467)/3  "CYBER_FAULT"
  App_Serv_1 (467)/1 -> L2S_1 (226)/1  "TLC_CONN"
  App_Serv_1 (467)/2 -> L2S_1 (226)/2  "TLC_SERVICE"
  App_Serv_1 (467)/3 -> L2S_1 (226)/3  "CYBER_FAULT"
  CISIA_MASTER (0)/2 -> Display19/1  "MAJOR HITS"
  CISIA_MASTER (0)/1 -> Display18/1  "MINOR HITS"
  CISIA_MASTER (0)/3 -> Display20/1  "DELTA TIME"
  CISIA_MASTER (0)/4 -> Display21/1  "TIME PAST"
